simulink library "outp"  (R2021b)
settings: Solver=VariableStepAuto  StartTime=0.0  StopTime=10.0  RelTol=1e-3
undefined symbols (not defined in the file or in its folder): ENUM_PMMMODE_CHARGE, ENUM_PMMMODE_IDLE, ENUM_PMMMODE_INITIALIZE, ENUM_PMMMODE_POWERDOWN, ENUM_PMMMODE_SLEEP, Left, outp, slcm, TRUE
libraries: FVT_lib x645, hcu_lib x4, simulink x1
(part 4 of 7)

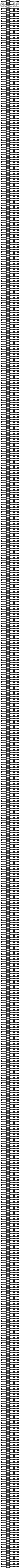
== system outp/OUTP/outpmodule ==
  VACC_HVTHCMSysAvail_enum : Inport
  VACC_LVBattVoltSta_enum : Inport  Port=2
  VACC_VehHVPwrAvail4THCM_W : Inport  Port=3
  VACC_EHPSEnDem_enum : Inport  Port=4
  VACC_CACPresWarnSta_flg : Inport  Port=5
  VACC_CACTempWarnSta_flg : Inport  Port=6
  VACC_EACEnDem_enum : Inport  Port=7
  VAPM_VehSpeedToAPM_kph : Inport  Port=8
  VAPM_VehSpeedTimeOut_flg : Inport  Port=9
  VAPM_FSOffSw_enum : Inport  Port=10
  VAPM_FSOffSwTimeOut_flg : Inport  Port=11
  VAPM_ChrgPlugSta_enum : Inport  Port=12
  VAPM_PASDRMR_cm : Inport  Port=13
  VAPM_PASDRML_cm : Inport  Port=14
  VAPM_PASDRCR_cm : Inport  Port=15
  VAPM_PASDRCL_cm : Inport  Port=16
  VAPM_PASDFMR_cm : Inport  Port=17
  VAPM_PASDFML_cm : Inport  Port=18
  VAPM_PASDFCR_cm : Inport  Port=19
  VAPM_PASDFCL_cm : Inport  Port=20
  VAPM_APSDRLR_cm : Inport  Port=21
  VAPM_APSDRLL_cm : Inport  Port=22
  VAPM_APSDFLR_cm : Inport  Port=23
  VAPM_APSDFLL_cm : Inport  Port=24
  VAPM_PASAFCL_enum : Inport  Port=25
  VAPM_PASARMR_enum : Inport  Port=26
  VAPM_PASARML_enum : Inport  Port=27
  VAPM_PASARCR_enum : Inport  Port=28
  VAPM_PASARCL_enum : Inport  Port=29
  VAPM_PASAFMR_enum : Inport  Port=30
  VAPM_PASAFML_enum : Inport  Port=31
  VAPM_PASAFCR_enum : Inport  Port=32
  VAPM_USSStaRMR_flg : Inport  Port=33
  VAPM_USSStaRML_flg : Inport  Port=34
  VAPM_USSStaRLR_flg : Inport  Port=35
  VAPM_USSStaRLL_flg : Inport  Port=36
  VAPM_USSStaRCR_flg : Inport  Port=37
  VAPM_USSStaRCL_flg : Inport  Port=38
  VAPM_USSStaFMR_flg : Inport  Port=39
  VAPM_USSStaFML_flg : Inport  Port=40
  VAPM_USSStaFLR_flg : Inport  Port=41
  VAPM_USSStaFLL_flg : Inport  Port=42
  VAPM_USSStaFCR_flg : Inport  Port=43
  VAPM_USSStaFCL_flg : Inport  Port=44
  VAPM_Chime_enum : Inport  Port=45
  VAPM_SNSRLayout_enum : Inport  Port=46
  VAPM_StaFSya_flg : Inport  Port=47
  VAPM_ModOperation_enum : Inport  Port=48
  VAPM_BrkPedalPosToAPM_pct : Inport  Port=49
  VAPM_BrkPedalPosTimeOut_flg : Inport  Port=50
  VAPM_LFRawWhlSpeed_kph : Inport  Port=51
  VAPM_LFRawWhlSpeedTimeOut_flg : Inport  Port=52
  VAPM_RFRawWhlSpeed_kph : Inport  Port=53
  VAPM_RFRawWhlSpeedTimeOut_flg : Inport  Port=54
  VAPM_LRRawWhlSpeed_kph : Inport  Port=55
  VAPM_LRRawWhlSpeedTimeOut_flg : Inport  Port=56
  VAPM_RRRawWhlSpeed_kph : Inport  Port=57
  VAPM_RRRawWhlSpeedTimeOut_flg : Inport  Port=58
  VAPM_LFRawWhlSpeedV_flg : Inport  Port=59
  VAPM_LFRawWhlSpeedVTimeOut_flg : Inport  Port=60
  VAPM_RFRawWhlSpeedV_flg : Inport  Port=61
  VAPM_RFRawWhlSpeedVTimeOut_flg : Inport  Port=62
  VAPM_LRRawWhlSpeedV_flg : Inport  Port=63
  VAPM_LRRawWhlSpeedVTimeOut_flg : Inport  Port=64
  VAPM_RRRawWhlSpeedV_flg : Inport  Port=65
  VAPM_RRRawWhlSpeedVTimeOut_flg : Inport  Port=66
  VAPM_LFWhlRotDir_enum : Inport  Port=67
  VAPM_LFWhlRotDirTimeOut_flg : Inport  Port=68
  VAPM_RFWhlRotDir_enum : Inport  Port=69
  VAPM_RFWhlRotDirTimeOut_flg : Inport  Port=70
  VAPM_LRWhlRotDir_enum : Inport  Port=71
  VAPM_LRWhlRotDirTimeOut_flg : Inport  Port=72
  VAPM_RRWhlRotDir_enum : Inport  Port=73
  VAPM_RRWhlRotDirTimeOut_flg : Inport  Port=74
  VAPM_LFPulseCountV_flg : Inport  Port=75
  VAPM_LFPulseCountVTimeOut_flg : Inport  Port=76
  VAPM_RFPulseCountV_flg : Inport  Port=77
  VAPM_RFPulseCountVTimeOut_flg : Inport  Port=78
  VAPM_LRPulseCountV_flg : Inport  Port=79
  VAPM_LRPulseCountVTimeOut_flg : Inport  Port=80
  VAPM_RRPulseCountV_flg : Inport  Port=81
  VAPM_RRPulseCountVTimeOut_flg : Inport  Port=82
  VAPM_LFPulseCount_enum : Inport  Port=83
  VAPM_LFPulseCountTimeOut_flg : Inport  Port=84
  VAPM_RFPulseCount_enum : Inport  Port=85
  VAPM_RFPulseCountTimeOut_flg : Inport  Port=86
  VAPM_LRPulseCount_enum : Inport  Port=87
  VAPM_LRPulseCountTimeOut_flg : Inport  Port=88
  VAPM_RRPulseCount_enum : Inport  Port=89
  VAPM_RRPulseCountTimeOut_flg : Inport  Port=90
  VAPM_ShifterHandleCmd_enum : Inport  Port=91
  VAPM_ShifterHandleCmdTimeOut_flg : Inport  Port=92
  VAPM_DriIntend_enum : Inport  Port=93
  VAPM_DriIntendTimeOut_flg : Inport  Port=94
  VAPM_EPSAOIControl_enum : Inport  Port=95
  VAPM_EPSAOIControlTimeOut_flg : Inport  Port=96
  VAPM_SASAngle_Deg : Inport  Port=97
  VAPM_SASAngleTimeOut_flg : Inport  Port=98
  VAPM_SASSpeed_degps : Inport  Port=99
  VAPM_SASSpeedTimeOut_flg : Inport  Port=100
  VAPM_SASSpeedValid_flg : Inport  Port=101
  VAPM_SASSpeedValidTimeOut_flg : Inport  Port=102
  VAPM_SASCAL_flg : Inport  Port=103
  VAPM_SASCALTimeOut_flg : Inport  Port=104
  VAPM_SASV_flg : Inport  Port=105
  VAPM_SASVTimeOut_flg : Inport  Port=106
  VAPM_GRADE_Deg : Inport  Port=107
  VAPM_GRADETimeOut_flg : Inport  Port=108
  VAPM_YawRate_degps : Inport  Port=109
  VAPM_YawRateTimeOut_flg : Inport  Port=110
  VAPM_LatAccel_Gps : Inport  Port=111
  VAPM_LatAccelTimeOut_flg : Inport  Port=112
  VAPM_LongAccel_Gps : Inport  Port=113
  VAPM_LongAccelTimeOut_flg : Inport  Port=114
  VAPM_MCPressure_bar : Inport  Port=115
  VAPM_MCPressureTimeOut_flg : Inport  Port=116
  VAPM_YawRateV_flg : Inport  Port=117
  VAPM_YawRateVTimeOut_flg : Inport  Port=118
  VAPM_LatAccelV_flg : Inport  Port=119
  VAPM_LatAccelVTimeOut_flg : Inport  Port=120
  VAPM_LongAccelV_flg : Inport  Port=121
  VAPM_LongAccelVTimeOut_flg : Inport  Port=122
  VAPM_MCPressureV_bar : Inport  Port=123
  VAPM_MCPressureVTimeOut_flg : Inport  Port=124
  VAPM_BrkSwSta_flg : Inport  Port=125
  VAPM_BrkSwStaTimeOut_flg : Inport  Port=126
  VAPM_BrkSwV_flg : Inport  Port=127
  VAPM_BrkSwVTimeOut_flg : Inport  Port=128
  VAPM_ESCStandstill_flg : Inport  Port=129
  VAPM_ESCStandstillTimeOut_flg : Inport  Port=130
  VAPM_ESCAPSSta_enum : Inport  Port=131
  VAPM_ESCAPSStaTimeOut_flg : Inport  Port=132
  VAPM_EPBExtReleaseAvail_flg : Inport  Port=133
  VAPM_EPBExtReleaseAvailTimeOut_flg : Inport  Port=134
  VAPM_EPBExtApplyAvail_flg : Inport  Port=135
  VAPM_EPBExtApplyAvailTimeOut_flg : Inport  Port=136
  VAPM_EPBErrSta_enum : Inport  Port=137
  VAPM_EPBErrStaTimeOut_flg : Inport  Port=138
  VAPM_EPBSta_enum : Inport  Port=139
  VAPM_EPBStaTimeOut_flg : Inport  Port=140
  VAPM_AVMparkingcancel_enum : Inport  Port=141
  VAPM_AVMparkingcancelTimeOut_flg : Inport  Port=142
  VAPM_AVMparkingexcute_enum : Inport  Port=143
  VAPM_AVMparkingexcuteTimeOut_flg : Inport  Port=144
  VAPM_AVMParkingmode_enum : Inport  Port=145
  VAPM_AVMParkingmodeTimeOut_flg : Inport  Port=146
  VAPM_AVMErrSTA_flg : Inport  Port=147
  VAPM_AVMErrSTATimeOut_flg : Inport  Port=148
  VAPM_IVIStatus_flg : Inport  Port=149
  VAPM_IVIStatusTimeOut_flg : Inport  Port=150
  VAPM_CAASSw_enum : Inport  Port=151
  VAPM_CAASSwTimeOut_flg : Inport  Port=152
  VAPM_IVIScreen_enum : Inport  Port=153
  VAPM_IVIScreenTimeOut_flg : Inport  Port=154
  VAPM_ABSActiveToAPM_flg : Inport  Port=155
  VAPM_ABSActiveTimeOut_flg : Inport  Port=156
  VAPM_TCSActiveToAPM_flg : Inport  Port=157
  VAPM_TCSActiveTimeOut_flg : Inport  Port=158
  VAPM_DriverSeatBeltCmd_flg : Inport  Port=159
  VAPM_DriverSeatBeltCmdTimeOut_flg : Inport  Port=160
  VAPM_APSProgressPCT_pct : Inport  Port=161
  VAPM_APSRQDisplay_enum : Inport  Port=162
  VAPM_APSSWVer_enum : Inport  Port=163
  VAPM_APSHWVer_enum : Inport  Port=164
  VAPM_APSExitCondition_enum : Inport  Port=165
  VAPM_APSAngleTarget_Deg : Inport  Port=166
  VAPM_APSVRqEPASCtrl_flg : Inport  Port=167
  VAPM_APSRqEPASCtrl_flg : Inport  Port=168
  VAPM_CAASSta_enum : Inport  Port=169
  VBCM_HornCtrl_flg : Inport  Port=170
  VBCM_FRHaltBrakeSta_enum : Inport  Port=171
  VBCM_FRDisIntEmCmd_flg : Inport  Port=172
  VBCM_FROpenClosePBCmd_enum : Inport  Port=173
  VBCM_DoorStaSta_enum : Inport  Port=174
  VBCM_BrakeLamp_flg : Inport  Port=175
  VBCM_LDRL_flg : Inport  Port=176
  VBCM_RDRL_flg : Inport  Port=177
  VBCM_ReverseLamp_flg : Inport  Port=178
  VBCM_RrFogLamp_flg : Inport  Port=179
  VBCM_HBeam_flg : Inport  Port=180
  VBCM_LBeam_flg : Inport  Port=181
  VBCM_PosLamp_flg : Inport  Port=182
  VBCM_HazardSW_flg : Inport  Port=183
  VBCM_LTurnLP_flg : Inport  Port=184
  VBCM_RTurnLP_flg : Inport  Port=185
  VBCM_LSMLPCmd_flg : Inport  Port=186
  VBCM_RSMLPCmd_flg : Inport  Port=187
  VBCM_TurnLpLActiveCmd_flg : Inport  Port=188
  VBCM_TurnLpRActiveCmd_flg : Inport  Port=189
  VBCM_BBuzzerCmd_flg : Inport  Port=190
  VBCM_FrWiperL_flg : Inport  Port=191
  VBCM_FrWiperH_flg : Inport  Port=192
  VBCM_WasherCtrl_enum : Inport  Port=193
  VBCM_RrRmLampBrightCmd_enum : Inport  Port=194
  VBCM_WelcomeDemoSta_flg : Inport  Port=195
  VBCM_FrAtmoLampCmd_flg : Inport  Port=196
  VBCM_RrAtmoLampCmd_flg : Inport  Port=197
  VBCM_TgateHDSWLSta_flg : Inport  Port=198
  VBCM_TgateHDSWRSta_flg : Inport  Port=199
  VBCM_TgateSWLSta_flg : Inport  Port=200
  VBCM_TgateSWRSta_flg : Inport  Port=201
  VBCM_LTgateRelCmd_flg : Inport  Port=202
  VBCM_RTgateRelCmd_flg : Inport  Port=203
  VBCM_FDDoorOpen_enum : Inport  Port=204
  VBCM_FDDoorstate_enum : Inport  Port=205
  VDHP_ActAPSPosn_pct : Inport  Port=206
  VDHP_EAPS1MIN_pct : Inport  Port=207
  VDHP_EAPS2MIN_pct : Inport  Port=208
  VDKC_DKCTimeSN_cnt : Inport  Port=209
  VDKC_DKCAuthSta_enum : Inport  Port=210
  VDSC_DISCTurn_flg : Inport  Port=211
  VDSC_DISCTargetSpd_kph : Inport  Port=212
  VDSC_DISCSta_enum : Inport  Port=213
  VDSC_DISCButtSta_flg : Inport  Port=214
  VNMM_AllCANTxReq_flg : Inport  Port=215
  VNMM_NMmTxReq_flg : Inport  Port=216
  VNMM_Awake_enum : Inport  Port=217
  VNMM_CSB_flg : Inport  Port=218
  VNMM_ErrorState_enum : Inport  Port=219
  VNMM_NodeID_enum : Inport  Port=220
  VNMM_PNI_flg : Inport  Port=221
  VNMM_RptMsgReq_flg : Inport  Port=222
  VNMM_WakeUp_enum : Inport  Port=223
  VNMM_ActiveWU_flg : Inport  Port=224
  VNMM_SysNMmSta_enum : Inport  Port=225
  VNMM_NetworkReq_flg : Inport  Port=226
  VPMM_PowerUpState_enum : Inport  Port=227
  VPMM_PowerDownState_enum : Inport  Port=228
  VPMM_PowerUpFault_enum : Inport  Port=229
  VPMM_PowerDownFault_enum : Inport  Port=230
  VPMM_ActiveDischargeReq_flg : Inport  Port=231
  VPMM_DCDCEnaReq_flg : Inport  Port=232
  VPMM_DCDCVoltSetpoint_V : Inport  Port=233
  VPMM_HVBatCnctReq_flg : Inport  Port=234
  VPMM_HVSysReadyToCharge_enum : Inport  Port=235
  VPMM_PowerSta_enum : Inport  Port=236
  VPMM_LVPwrSta_flg : Inport  Port=237
  VPMM_HVPwrSta_flg : Inport  Port=238
  VPMM_SysPowerMode_enum : Inport  Port=239
  VPMM_FrMCUEnaReq_flg : Inport  Port=240
  VPMM_RrMCUEnaReq_flg : Inport  Port=241
  VPMM_DrivetrainSelect_enum : Inport  Port=242
  VPMM_DrSeatSta_enum : Inport  Port=243
  VPMM_PwrStaSelect_enum : Inport  Port=244
  VPMM_PwrStaConstraint_enum : Inport  Port=245
  VPMM_TCountSta_enum : Inport  Port=246
  VPMM_PwrUpReq_enum : Inport  Port=247
  VPMM_PwrDownReq_enum : Inport  Port=248
  VPMM_LowSOCWarn_enum : Inport  Port=249
  VPMM_ReVehThdChkSta_enum : Inport  Port=250
  VPMM_LVSysErrPwrOutErr_flg : Inport  Port=251
  VPMM_EvccAplusPwrUpReq_flg : Inport  Port=252
  VPMM_PwrStaONTOPopReq_flg : Inport  Port=253
  VPMM_IVIPwrStaONTOPopT_s : Inport  Port=254
  VPMM_LVChrgHoldTtimer_s : Inport  Port=255
  VPMM_LVBattChrgTimeCnt_s : Inport  Port=256
  VPMM_SilentChkAllowSleep_flg : Inport  Port=257
  VPMM_TimerAllowSleep_flg : Inport  Port=258
  VPMM_FDADC12VDetAvg_mV : Inport  Port=259
  VPMM_PMMAllowECUSleep_flg : Inport  Port=260
  VPMM_LVSilentChrgSta_enum : Inport  Port=261
  VPMM_LVSilentChrgReq_flg : Inport  Port=262
  VPMM_LVSilentChrgLv_enum : Inport  Port=263
  VPMM_CtrlFrPwrStbA1P_flg : Inport  Port=264
  VPMM_CtrlFrRC1_flg : Inport  Port=265
  VPMM_CtrlFrBMSCCUCIR_flg : Inport  Port=266
  VPMM_CtrlFrEDUINVERTER_flg : Inport  Port=267
  VPMM_HWResetSta_enum : Inport  Port=268
  VPMM_CtrlDrPwrStbA2_flg : Inport  Port=269
  VPMM_PwrStaTOSta_enum : Inport  Port=270
  VPMM_DCDCRlyDem_enum : Inport  Port=271
  VPMM_EACRlyDem_enum : Inport  Port=272
  VPMM_EHPSRlyDem_enum : Inport  Port=273
  VPMM_DCDCEnDem_enum : Inport  Port=274
  VSCP_Vehspeed_kph : Inport  Port=275
  VSCP_SCPBrkSwSta_flg : Inport  Port=276
  VSCP_AmberWnlmpSta_flg : Inport  Port=277
  VSCP_ABSWnlmpSta_flg : Inport  Port=278
  VSCP_HSAFailed_flg : Inport  Port=279
  VSCP_MeterIndVehSpeed_kph : Inport  Port=280
  VSCP_ABSFailed_flg : Inport  Port=281
  VSCP_ABSActive_flg : Inport  Port=282
  VSCP_HSAActive_flg : Inport  Port=283
  VSCP_RedWnlmpSta_flg : Inport  Port=284
  VSCP_BrkPedalPos_pct : Inport  Port=285
  VSCP_OpenStatusOfDoor1_enum : Inport  Port=286
  VSCP_OpenStatusOfDoor2_enum : Inport  Port=287
  VSCP_SeatBeltSwitch_enum : Inport  Port=288
  VSCP_triggerBAM_flg : Inport  Port=289
  VSCP_CFGEM1Ctrl_raw : Inport  Port=290
  VSCP_CFGEM1BAMTSize_raw : Inport  Port=291
  VSCP_CFGEM1BAMTNum_raw : Inport  Port=292
  VSCP_CFGEM1BAMRsv_raw : Inport  Port=293
  VSCP_CFGEM1BAMPGN_raw : Inport  Port=294
  VSCP_triggerDT_flg : Inport  Port=295
  VSCP_DTbyte0_raw : Inport  Port=296
  VSCP_DTbyte1_raw : Inport  Port=297
  VSCP_DTbyte2_raw : Inport  Port=298
  VSCP_DTbyte3_raw : Inport  Port=299
  VSCP_DTbyte4_raw : Inport  Port=300
  VSCP_DTbyte5_raw : Inport  Port=301
  VSCP_DTbyte6_raw : Inport  Port=302
  VSCP_DTbyte7_raw : Inport  Port=303
  VSYS_HWVer1_cnt : Inport  Port=304
  VSYS_HWVer2_cnt : Inport  Port=305
  VSYS_HWVer3_cnt : Inport  Port=306
  VSYS_CarModel1_cnt : Inport  Port=307
  VSYS_CarModel2_cnt : Inport  Port=308
  VSYS_CarModel3_cnt : Inport  Port=309
  VSYS_ECU1_cnt : Inport  Port=310
  VSYS_ECU2_cnt : Inport  Port=311
  VSYS_Major1_cnt : Inport  Port=312
  VSYS_Major2_cnt : Inport  Port=313
  VSYS_Minor1_cnt : Inport  Port=314
  VSYS_Minor2_cnt : Inport  Port=315
  VSYS_Patch1_cnt : Inport  Port=316
  VSYS_Patch2_cnt : Inport  Port=317
  VSYS_Country1_cnt : Inport  Port=318
  VSYS_Country2_cnt : Inport  Port=319
  VSYS_Variation_cnt : Inport  Port=320
  VSYS_Dash1_cnt : Inport  Port=321
  VSYS_Change1_cnt : Inport  Port=322
  VSYS_Change2_cnt : Inport  Port=323
  VSYS_Dash2_cnt : Inport  Port=324
  VSYS_SHA1_cnt : Inport  Port=325
  VSYS_SHA2_cnt : Inport  Port=326
  VSYS_SHA3_cnt : Inport  Port=327
  VSYS_SHA4_cnt : Inport  Port=328
  VSYS_SHA5_cnt : Inport  Port=329
  VSYS_SHA6_cnt : Inport  Port=330
  VSYS_SHA7_cnt : Inport  Port=331
  VSYS_SHA8_cnt : Inport  Port=332
  VSYS_NvWriteReqRisingEdge_flg : Inport  Port=333
  VSYS_FdcSlpReqRisingEdge_flg : Inport  Port=334
  VSYS_FdcSlpTime_sec : Inport  Port=335
  VSYS_PmicBootReason_enum : Inport  Port=336
  VSYS_WisrBootReason_raw32 : Inport  Port=337
  VSYS_AcoreRebootCmdACK_flg : Inport  Port=338
  VSYS_CurrentNmState_enum : Inport  Port=339
  VTHC_FDCompCmd_rpm : Inport  Port=340
  VTHC_FDSOV1Cmd_flg : Inport  Port=341
  VTHC_FDSOV2Cmd_flg : Inport  Port=342
  VTHC_FDSOV3Cmd_flg : Inport  Port=343
  VTHC_FDEXV1Cmd_step : Inport  Port=344
  VTHC_FDEXV2Cmd_step : Inport  Port=345
  VTHC_FDSOTXVCmd_flg : Inport  Port=346
  VTHC_FDFWVCmd_flg : Inport  Port=347
  VTHC_FDTWVCmd_pct : Inport  Port=348
  VTHC_FDFrWPTCHeatPwrCmd_W : Inport  Port=349
  VTHC_CoolgFanActDuty_pct : Inport  Port=350
  VTHC_FDAGSCmd_enum : Inport  Port=351
  VTHC_FDEWP1Cmd_enum : Inport  Port=352
  VTHC_FDEWP2Cmd_enum : Inport  Port=353
  VTHC_FDEWP3Cmd_enum : Inport  Port=354
  VTHC_FDFrLeAPTCHeatPwrCmd_W : Inport  Port=355
  VTHC_FDFrRiAPTCHeatPwrCmd_W : Inport  Port=356
  VTHC_FDRrAPTCHeatPwrCmd_W : Inport  Port=357
  VTHC_FDBlowerCmd_pct : Inport  Port=358
  VTHC_BatteryMode_enum : Inport  Port=359
  VTHC_EDriveMode_enum : Inport  Port=360
  VTHC_CabinMode_enum : Inport  Port=361
  VTHC_CCUACLampSts_flg : Inport  Port=362
  VTHC_CCUAutoLampSts_flg : Inport  Port=363
  VTHC_CCUACMaxLampSts_flg : Inport  Port=364
  VTHC_CCUSyncLampSts_flg : Inport  Port=365
  VTHC_sigAirIntenZon1St_enum : Inport  Port=366
  VTHC_sigWindDirZon1St_enum : Inport  Port=367
  VTHC_sigRecircSt_flg : Inport  Port=368
  VTHC_sigSetTempZon1St_C : Inport  Port=369
  VTHC_sigSetTempZon2St_C : Inport  Port=370
  VTHC_sigClntTHvBattOut_C : Inport  Port=371
  VTHC_sigCbnSolarLeft_W : Inport  Port=372
  VTHC_sigClntTHvBattIn_C : Inport  Port=373
  VTHC_sigCbnSolarRight_W : Inport  Port=374
  VTHC_sigAmbAirT_C : Inport  Port=375
  VTHC_sigCbnAirT_C : Inport  Port=376
  VTHC_ACSubMode_enum : Inport  Port=377
  VTHC_FDRecyAutoCmd_enum : Inport  Port=378
  VTHC_ACModeMem_enum : Inport  Port=379
  VTHC_Face_flg : Inport  Port=380
  VTHC_Foot_flg : Inport  Port=381
  VTHC_Frost_flg : Inport  Port=382
  VTHC_FaceM_flg : Inport  Port=383
  VTHC_FootM_flg : Inport  Port=384
  VTHC_CCUSyncSts_flg : Inport  Port=385
  VTHC_ACForceOFF_flg : Inport  Port=386
  VTHC_RecAutoFlg_flg : Inport  Port=387
  VTHC_AirIntenZone1M_enum : Inport  Port=388
  VTHC_fdefog_flg : Inport  Port=389
  VTHC_sigSetTempZon2StM_C : Inport  Port=390
  VTHC_FDCTHCMAPTCWarningSta_flg : Inport  Port=391
  VTPM_LFBatWarn_flg : Inport  Port=392
  VTPM_RFBatWarn_flg : Inport  Port=393
  VTPM_LRBatWarn_flg : Inport  Port=394
  VTPM_RRBatWarn_flg : Inport  Port=395
  VTPM_LFWheelPress_raw8 : Inport  Port=396
  VTPM_RFWheelPress_raw8 : Inport  Port=397
  VTPM_LRWheelPress_raw8 : Inport  Port=398
  VTPM_RRWheelPress_raw8 : Inport  Port=399
  VTPM_LFWheelTemp_C : Inport  Port=400
  VTPM_RFWheelTemp_C : Inport  Port=401
  VTPM_LRWheelTemp_C : Inport  Port=402
  VTPM_RRWheelTemp_C : Inport  Port=403
  VTPM_LFSensorFail_flg : Inport  Port=404
  VTPM_RFSensorFail_flg : Inport  Port=405
  VTPM_LRSensorFail_flg : Inport  Port=406
  VTPM_RRSensorFail_flg : Inport  Port=407
  VTPM_LFWheelDebug_flg : Inport  Port=408
  VTPM_LRWheelDebug_flg : Inport  Port=409
  VTPM_RFWheelDebug_flg : Inport  Port=410
  VTPM_RRWheelDebug_flg : Inport  Port=411
  VTPM_TPMSResButtAllow_flg : Inport  Port=412
  VTPM_TPMSCaliButtAllow_flg : Inport  Port=413
  VTPM_LFPressIndi_enum : Inport  Port=414
  VTPM_RFPressIndi_enum : Inport  Port=415
  VTPM_LRPressIndi_enum : Inport  Port=416
  VTPM_RRPressIndi_enum : Inport  Port=417
  VTPM_TPMSWarnIndi_enum : Inport  Port=418
  VTPM_LFWheelTmpIndi_flg : Inport  Port=419
  VTPM_RFWheelTmpIndi_flg : Inport  Port=420
  VTPM_LRWheelTmpIndi_flg : Inport  Port=421
  VTPM_RRWheelTmpIndi_flg : Inport  Port=422
  VTPM_LFWheelPSW_raw8 : Inport  Port=423
  VTPM_LRWheelPSW_raw8 : Inport  Port=424
  VTPM_RFWheelPSW_raw8 : Inport  Port=425
  VTPM_RRWheelPSW_raw8 : Inport  Port=426
  VTPM_CWheelTips_enum : Inport  Port=427
  VTPM_AutoLTips_enum : Inport  Port=428
  VTPM_LFSensorMode_flg : Inport  Port=429
  VTPM_RFSensorMode_flg : Inport  Port=430
  VTPM_LRSensorMode_flg : Inport  Port=431
  VTPM_RRSensorMode_flg : Inport  Port=432
  VTPM_S1ID_raw32 : Inport  Port=433
  VTPM_S2ID_raw32 : Inport  Port=434
  VTPM_S3ID_raw32 : Inport  Port=435
  VTPM_S4ID_raw32 : Inport  Port=436
  VTPM_S1L_enum : Inport  Port=437
  VTPM_S2L_enum : Inport  Port=438
  VTPM_S3L_enum : Inport  Port=439
  VTPM_S4L_enum : Inport  Port=440
  VTPM_ALFin_flg : Inport  Port=441
  VTPM_LFP20_raw8 : Inport  Port=442
  VTPM_RFP20_raw8 : Inport  Port=443
  VTPM_LRP20_raw8 : Inport  Port=444
  VTPM_RRP20_raw8 : Inport  Port=445
  VTPM_FAT_flg : Inport  Port=446
  VTPM_IDin_raw32 : Inport  Port=447
  VTPM_S1WheelDebugALTU_pct : Inport  Port=448
  VTPM_S2WheelDebugALTU_pct : Inport  Port=449
  VTPM_S3WheelDebugALTU_pct : Inport  Port=450
  VTPM_S4WheelDebugALTU_pct : Inport  Port=451
  VTPM_ID1messageALTU_raw8 : Inport  Port=452
  VTPM_ID2messageALTU_raw8 : Inport  Port=453
  VTPM_ID3messageALTU_raw8 : Inport  Port=454
  VTPM_ID4messageALTU_raw8 : Inport  Port=455
  VTPM_Chkfin_flg : Inport  Port=456
  VTPM_SetIDLoc_flg : Inport  Port=457
  VTPM_TPMSStorge_flg : Inport  Port=458
  VTPM_ChkStorge_flg : Inport  Port=459
  VTPM_TPMSResButt_flg : Inport  Port=460
  VTPM_LFPindi_enum : Inport  Port=461
  VTPM_RFPind_enum : Inport  Port=462
  VTPM_LRPindi_enum : Inport  Port=463
  VTPM_RRPindi_enum : Inport  Port=464
  VTPM_WriteChkLFID_raw : Inport  Port=465
  VTPM_WriteChkRFID_raw : Inport  Port=466
  VTPM_WriteChkLRID_raw : Inport  Port=467
  VTPM_WriteChkRRID_raw : Inport  Port=468
  VTPM_WriteChkfinLFID_raw : Inport  Port=469
  VTPM_WriteChkfinRFID_raw : Inport  Port=470
  VTPM_WriteChkfinLRID_raw : Inport  Port=471
  VTPM_WriteChkfinRRID_raw : Inport  Port=472
  VTPM_Flashchkdatavalid_enum : Inport  Port=473
  VTPM_Flashdatavalid_enum : Inport  Port=474
  VTPM_unlearnSfali_flg : Inport  Port=475
  VTPM_unlearnSfailvalid_enum : Inport  Port=476
  VTPM_Prepresstempvalid_enum : Inport  Port=477
  VTPM_FlashS1ID_raw : Inport  Port=478
  VTPM_FlashS2ID_raw : Inport  Port=479
  VTPM_FlashS3ID_raw : Inport  Port=480
  VTPM_FlashS4ID_raw : Inport  Port=481
  VTPM_FlashIDvalid_enum : Inport  Port=482
  VTQD_ParkRequest_flg : Inport  Port=483
  VTQD_TqSourceFr_enum : Inport  Port=484
  VTQD_TqSourceRr_enum : Inport  Port=485
  VTQD_FrEDUAvailBrkRgnTq_Nm : Inport  Port=486
  VTQD_RrEDUAvailBrkRgnTq_Nm : Inport  Port=487
  VTQD_EVDriveMode_enum : Inport  Port=488
  VTQD_ShiftGearPosn_enum : Inport  Port=489
  VTQD_PButtonSta_enum : Inport  Port=490
  VTQD_FrActvDmpDisabReq_flg : Inport  Port=491
  VTQD_RrActvDmpDisabReq_flg : Inport  Port=492
  VTQD_FrRgnDecrSta_flg : Inport  Port=493
  VTQD_RrRgnDecrSta_flg : Inport  Port=494
  VTQD_DriverWhlTqDemFr_Nm : Inport  Port=495
  VTQD_DriverWhlTqDemRr_Nm : Inport  Port=496
  VTQD_FrEDUActTq_Nm : Inport  Port=497
  VTQD_RrEDUActTq_Nm : Inport  Port=498
  VTQD_FrEDURolRgnTq_Nm : Inport  Port=499
  VTQD_RrEDURolRgnTq_Nm : Inport  Port=500
  VTQD_FrEDUSpd_rpm : Inport  Port=501
  VTQD_RrEDUSpd_rpm : Inport  Port=502
  VTQD_FrEDUSpdValid_flg : Inport  Port=503
  VTQD_FrEDUAvailBrkRgnTqV_flg : Inport  Port=504
  VTQD_RrEDUSpdValid_flg : Inport  Port=505
  VTQD_RrEDUAvailBrkRgnTqV_flg : Inport  Port=506
  VTQD_RgnAbnorSta_flg : Inport  Port=507
  VTQD_PTCSPermSta_flg : Inport  Port=508
  VTQD_FrRgnPermSta_flg : Inport  Port=509
  VTQD_RrRgnPermSta_flg : Inport  Port=510
  VTQD_FrIdcMin_A : Inport  Port=511
  VTQD_FrIdcMax_A : Inport  Port=512
  VTQD_FrUdcMin_V : Inport  Port=513
  VTQD_FrUdcMax_V : Inport  Port=514
  VTQD_RrIdcMin_A : Inport  Port=515
  VTQD_RrIdcMax_A : Inport  Port=516
  VTQD_RrUdcMin_V : Inport  Port=517
  VTQD_RrUdcMax_V : Inport  Port=518
  VTQD_ReBrakeLPReq_flg : Inport  Port=519
  VTQD_CreepON_flg : Inport  Port=520
  VTQD_ActEMpTrq_pct : Inport  Port=521
  VTQD_ActMaxAvaEMRecpTrq_pct : Inport  Port=522
  VTQD_ActDriveDirect_enum : Inport  Port=523
  VTQD_DLEngaged_enum : Inport  Port=524
  VTQD_EMTrqModeDrvBrk_enum : Inport  Port=525
  VTQD_ActEMpTrqHrls_pct : Inport  Port=526
  VTQD_ActEMOutSftSpd_rpm : Inport  Port=527
  VTQD_DrvDemEMRtapTrq_pct : Inport  Port=528
  VTQD_SACtrlDev_enum : Inport  Port=529
  VTQD_RetSelNonEng_pct : Inport  Port=530
  VTQD_ShiftPgs_enum : Inport  Port=531
  VTQD_AccPedal1LowSW_enum : Inport  Port=532
  VTQD_AccPedalPos1_pct : Inport  Port=533
  VTQD_ParkBrakeSW_enum : Inport  Port=534
  VTQD_VCUVehSpd_kph : Inport  Port=535
  VTQD_BrakeSW_enum : Inport  Port=536
  VTQD_NFricPercTorq_pct : Inport  Port=537
  VTQD_EMParasLoss_pct : Inport  Port=538
  VTQD_EEC2MSGCnt_raw : Inport  Port=539
  VTQD_EEC2MSGCS_raw : Inport  Port=540
  VTQD_FDCCHAEBSRd4BRSta_enum : Inport  Port=541
  VTQD_FDCCHAEBSHBSwSta_enum : Inport  Port=542
  VTQD_FDCCHAEBSHHSwSta_enum : Inport  Port=543
  VTQD_FDCVCUTUpAStaSta_enum : Inport  Port=544
  VTQD_FDCVCUDACStatusSta_enum : Inport  Port=545
  VTQR_FrTMTqReq_Nm : Inport  Port=546
  VTQR_RrTMTqReq_Nm : Inport  Port=547
  VV2L_ReqOBCV2LEna_enum : Inport  Port=548
  VV2L_ReqV2LIVIPopup_enum : Inport  Port=549
  VVMC_FeatSetSpdFinal_raw32 : Inport  Port=550
  VVMC_VehicleSpeed_mph : Inport  Port=551
  VVMC_VehicleSpeed_kph : Inport  Port=552
  VVMC_MeterIndSpeed_raw32 : Inport  Port=553
  VVMC_VMCAEBCtrlAvail_flg : Inport  Port=554
  VVMC_VMCACCCtrlAvail_flg : Inport  Port=555
  VVMC_VMCCCCtrlAvail_flg : Inport  Port=556
  VVMC_VMCMSACtrlAvail_flg : Inport  Port=557
  VVMC_FeatArbitrSta_enum : Inport  Port=558
  VVMC_FeatReqSpd_kph : Inport  Port=559
  VVMC_JerkPCT_pct : Inport  Port=560
  VVMC_LimitPCT_pct : Inport  Port=561
  VVMC_FrontRearSlipRatioCtrl_flg : Inport  Port=562
  VVMC_RearWhlSlipRatioCtrl_flg : Inport  Port=563
  VVMC_SingleWhlSlipRatioCtrl_flg : Inport  Port=564
  VVMC_LatAccCtrl_flg : Inport  Port=565
  VVMC_SafetyCtrl_flg : Inport  Port=566
  VVMC_SPD2ACCAct_flg : Inport  Port=567
  VVMC_AccCalcuPID_mps2 : Inport  Port=568
  VVMC_ISOAccLimit_mps2 : Inport  Port=569
  VVMC_ISODecLimit_mps2 : Inport  Port=570
  VVMC_ISOJerkLimit_mps3 : Inport  Port=571
  VVMC_ACCRequiredAccel_mps2 : Inport  Port=572
  VVMC_DISCReqAcc_mps2 : Inport  Port=573
  VVMC_FeatArbitrFinal_enum : Inport  Port=574
  VVMC_LateralCtrl_flg : Inport  Port=575
  VVMC_ADASLKASta_enum : Inport  Port=576
  VVMC_LKAStrToqReq_Nm : Inport  Port=577
  VVMC_LKATOIFault_flg : Inport  Port=578
  VVMC_LKATOIAct_enum : Inport  Port=579
  VVMC_ADASAEBReq_enum : Inport  Port=580
  VVMC_ADASFaultSta_flg : Inport  Port=581
  VVMC_AEBVehHoldReq_flg : Inport  Port=582
  VVMC_ACCVehHoldReq_flg : Inport  Port=583
  VVMC_ADASDBSReq_enum : Inport  Port=584
  VVMC_ADASACCSta_enum : Inport  Port=585
  VVMC_ACCObjDist_m : Inport  Port=586
  VVMC_ACCObjRelSpd_mps : Inport  Port=587
  VVMC_TimeGapLevel_enum : Inport  Port=588
  VVMC_ACCJerkUpperLimit_mps3 : Inport  Port=589
  VVMC_ACCComfortBandUpper_mps2 : Inport  Port=590
  VVMC_ACCJerkLowerLimit_mps3 : Inport  Port=591
  VVMC_ACCComfortBandLower_mps2 : Inport  Port=592
  VVMC_ADASVehSpdLim_raw32 : Inport  Port=593
  VVMC_ADASShftPosnReqA_flg : Inport  Port=594
  VVMC_ADASShftPosnReq_enum : Inport  Port=595
  VVMC_ADASForceIdle_flg : Inport  Port=596
  VVMC_HazardWarningReq_flg : Inport  Port=597
  VVMC_RightTurnLightReq_flg : Inport  Port=598
  VVMC_LeftTurnLightReq_flg : Inport  Port=599
  VVMC_ADASFCWSta_enum : Inport  Port=600
  VVMC_ADASLDWSta_enum : Inport  Port=601
  VVMC_ADASFltWrnReq_flg : Inport  Port=602
  VVMC_ACCObjDstLvl_enum : Inport  Port=603
  VVMC_ForceLowBeam_enum : Inport  Port=604
  VVMC_ACCTakeoverReq_flg : Inport  Port=605
  VVMC_ADASWarningMsg_enum : Inport  Port=606
  VVMC_ADASCAMSpdLim_enum : Inport  Port=607
  VVMC_TargetType_enum : Inport  Port=608
  VVMC_ADASSLIFSpdLim_enum : Inport  Port=609
  VVMC_LKAHODDisplayWarning_flg : Inport  Port=610
  VVMC_LKAHODSoundWarning_flg : Inport  Port=611
  VVMC_ADASLFCSta_enum : Inport  Port=612
  VVMC_ADASLaneModeL_enum : Inport  Port=613
  VVMC_ADASLaneModeR_enum : Inport  Port=614
  VVMC_ADASSLIFSta_enum : Inport  Port=615
  VVMC_ADASISASta_enum : Inport  Port=616
  VVMC_ADASLDWMute_flg : Inport  Port=617
  VVMC_ADASFCWMute_flg : Inport  Port=618
  VVMC_ADASLFCHandsOffWarning_enum : Inport  Port=619
  VVMC_LVDADisabled_flg : Inport  Port=620
  VVMC_LVDAMuteSta_enum : Inport  Port=621
  VVMC_LVDAFailinfo_flg : Inport  Port=622
  VVMC_LVDAWarning_flg : Inport  Port=623
  VVMC_LVDAACCStatusInformation_flg : Inport  Port=624
  VVMC_ADASLFCWarnSound_enum : Inport  Port=625
  VVMC_FCMACCmode_enum : Inport  Port=626
  VVMC_ADASLanetypeR_enum : Inport  Port=627
  VVMC_ADASLanetypeL_enum : Inport  Port=628
  VVMC_ADASLanecurveL_raw32 : Inport  Port=629
  VVMC_ADASLanecurveR_raw32 : Inport  Port=630
  VVMC_ADASAEBSta_enum : Inport  Port=631
  VVMC_FCMLDWRequest_enum : Inport  Port=632
  VVMC_FCMLDWFault_flg : Inport  Port=633
  VVMC_ACCCtrlAvail_flg : Inport  Port=634
  VVMC_ACCPedalOvrd_flg : Inport  Port=635
  VVMC_TimeGapCalcu_s : Inport  Port=636
  VVMC_CCCtrlSta_enum : Inport  Port=637
  VVMC_MSACtrlSta_enum : Inport  Port=638
  VVMC_APSCtrlAvail_flg : Inport  Port=639
  VVMC_APSStaSys_enum : Inport  Port=640
  VVMC_APSDecReqA_flg : Inport  Port=641
  VVMC_APSDecReq_mps2 : Inport  Port=642
  VVMC_APSReq_enum : Inport  Port=643
  VVMC_CCMSASpdWar_flg : Inport  Port=644
  VVMC_IMUEnaCmd_flg : Inport  Port=645
  UnitConverter{1..2,4,7,10,12..20,25..32,45..46,48,67,69,71,73,83,85,87,89,91,93,95,131,137,139,141,143,145,151,153,162..165,169,171,173..174,193..194,204..205,210,213,217,219..220,223,225,227..230,235..236,239,242..250,261,263,268,270..274,286..288,290,292..293,296..332,336,339,351..354,359..361,366..367,377..379,388,396..399,414..418,423..428,437..440,442..445,452..455,461..464,473..474,476..477,482,484..485,488..490,524..525,529,531..532,534,536,539..545,548..549,558,574,576,579..580,584..585,588,595,600..601,603..604,606..609,612..616,619,621,625..628,631..632,637..638,640,643} (236 alike) : DataTypeConversion  OutDataTypeStr=uint8
  UnitConverter{5..6,9,11,33..44,47,50,52,54,56,58..66,68,70,72,74..82,84,86,88,90,92,94,96,98,100..106,108,110,112,114,116..130,132..136,138,140,142,144,146..150,152,154..160,167..168,170,172,175..192,195..203,211,214..216,218,221..222,224,226,231..232,234,237..238,240..241,251..253,257..258,260,262,264..267,269,276..279,281..284,289,295,333..334,338,341..343,346..347,362..365,368,380..387,389,391..395,404..413,419..422,429..432,441,446,456..460,475,483,491..494,503..510,519..520,554..557,562..567,575,578,581..583,594,596..599,602,605,610..611,617..618,620,622..624,633..635,639,641,644..645} (272 alike) : DataTypeConversion  OutDataTypeStr=boolean
  UnitConverter{3,8,49,51,53,55,57,97,99,107,109,111,113,115,161,166,206..208,212,233,254..256,259,275,280,285,335,348..350,355..358,369..376,390,400..403,448..451,486..487,495..502,511..518,521..523,526..528,530,533,535,537..538,546..547,550..553,559..561,568..573,577,586..587,589..593,629..630,636,642} (109 alike) : DataTypeConversion  OutDataTypeStr=single
  UnitConverter{209,294,337,433..436,447,465..472,478..481} (20 alike) : DataTypeConversion  OutDataTypeStr=uint32
  UnitConverter{21..24,291,340,344..345} (8 alike) : DataTypeConversion  OutDataTypeStr=uint16
  VACC_CACPresWarnSta_flg_Inproc : FVT_lib/outp/OverrideAndLimit  SystemSampleTime=-1  VariantActivationTime=update diagram  Latency=0  AutoFrameSizeCalculation=off
      link override Signal_Limit/_maxval: Value=KOUTP_CACPresWarnSta_flg_maxval
      link override Signal_Limit/_minval: Value=KOUTP_CACPresWarnSta_flg_minval
      link override Signal_Override/_ovrdflg: Value=KOUTP_CACPresWarnSta_flg_ovrdflg
      link override Signal_Override/_ovrdval: Value=KOUTP_CACPresWarnSta_flg_ovrdval
  VACC_CACTempWarnSta_flg_Inproc : FVT_lib/outp/OverrideAndLimit  SystemSampleTime=-1  VariantActivationTime=update diagram  Latency=0  AutoFrameSizeCalculation=off
      link override Signal_Limit/_maxval: Value=KOUTP_CACTempWarnSta_flg_maxval
      link override Signal_Limit/_minval: Value=KOUTP_CACTempWarnSta_flg_minval
      link override Signal_Override/_ovrdflg: Value=KOUTP_CACTempWarnSta_flg_ovrdflg
      link override Signal_Override/_ovrdval: Value=KOUTP_CACTempWarnSta_flg_ovrdval
  VACC_EACEnDem_enum_Inproc : FVT_lib/outp/OverrideAndLimit  SystemSampleTime=-1  VariantActivationTime=update diagram  Latency=0  AutoFrameSizeCalculation=off
      link override Signal_Limit/_maxval: Value=KOUTP_EACEnDem_enum_maxval
      link override Signal_Limit/_minval: Value=KOUTP_EACEnDem_enum_minval
      link override Signal_Override/_ovrdflg: Value=KOUTP_EACEnDem_enum_ovrdflg
      link override Signal_Override/_ovrdval: Value=KOUTP_EACEnDem_enum_ovrdval
  VACC_EHPSEnDem_enum_Inproc : FVT_lib/outp/OverrideAndLimit  SystemSampleTime=-1  VariantActivationTime=update diagram  Latency=0  AutoFrameSizeCalculation=off
      link override Signal_Limit/_maxval: Value=KOUTP_EHPSEnDem_enum_maxval
      link override Signal_Limit/_minval: Value=KOUTP_EHPSEnDem_enum_minval
      link override Signal_Override/_ovrdflg: Value=KOUTP_EHPSEnDem_enum_ovrdflg
      link override Signal_Override/_ovrdval: Value=KOUTP_EHPSEnDem_enum_ovrdval
  VACC_HVTHCMSysAvail_enum_Inproc : FVT_lib/outp/OverrideAndLimit  SystemSampleTime=-1  VariantActivationTime=update diagram  Latency=0  AutoFrameSizeCalculation=off
      link override Signal_Limit/_maxval: Value=KOUTP_HVTHCMSysAvail_enum_maxval
      link override Signal_Limit/_minval: Value=KOUTP_HVTHCMSysAvail_enum_minval
      link override Signal_Override/_ovrdflg: Value=KOUTP_HVTHCMSysAvail_enum_ovrdflg
      link override Signal_Override/_ovrdval: Value=KOUTP_HVTHCMSysAvail_enum_ovrdval
  VACC_LVBattVoltSta_enum_Inproc : FVT_lib/outp/OverrideAndLimit  SystemSampleTime=-1  VariantActivationTime=update diagram  Latency=0  AutoFrameSizeCalculation=off
      link override Signal_Limit/_maxval: Value=KOUTP_LVBattVoltSta_enum_maxval
      link override Signal_Limit/_minval: Value=KOUTP_LVBattVoltSta_enum_minval
      link override Signal_Override/_ovrdflg: Value=KOUTP_LVBattVoltSta_enum_ovrdflg
      link override Signal_Override/_ovrdval: Value=KOUTP_LVBattVoltSta_enum_ovrdval
  VACC_VehHVPwrAvail4THCM_W_Inproc : FVT_lib/outp/OverrideAndLimit  SystemSampleTime=-1  VariantActivationTime=update diagram  Latency=0  AutoFrameSizeCalculation=off
      link override Signal_Limit/_maxval: Value=KOUTP_VehHVPwrAvail4THCM_W_maxval
      link override Signal_Limit/_minval: Value=KOUTP_VehHVPwrAvail4THCM_W_minval
      link override Signal_Override/_ovrdflg: Value=KOUTP_VehHVPwrAvail4THCM_W_ovrdflg
      link override Signal_Override/_ovrdval: Value=KOUTP_VehHVPwrAvail4THCM_W_ovrdval
  VAPM_ABSActiveTimeOut_flg_Inproc : FVT_lib/outp/OverrideAndLimit  SystemSampleTime=-1  VariantActivationTime=update diagram  Latency=0  AutoFrameSizeCalculation=off
      link override Signal_Limit/_maxval: Value=KOUTP_ABSActiveTimeOut_flg_maxval
      link override Signal_Limit/_minval: Value=KOUTP_ABSActiveTimeOut_flg_minval
      link override Signal_Override/_ovrdflg: Value=KOUTP_ABSActiveTimeOut_flg_ovrdflg
      link override Signal_Override/_ovrdval: Value=KOUTP_ABSActiveTimeOut_flg_ovrdval
  VAPM_ABSActiveToAPM_flg_Inproc : FVT_lib/outp/OverrideAndLimit  SystemSampleTime=-1  VariantActivationTime=update diagram  Latency=0  AutoFrameSizeCalculation=off
      link override Signal_Limit/_maxval: Value=KOUTP_ABSActiveToAPM_flg_maxval
      link override Signal_Limit/_minval: Value=KOUTP_ABSActiveToAPM_flg_minval
      link override Signal_Override/_ovrdflg: Value=KOUTP_ABSActiveToAPM_flg_ovrdflg
      link override Signal_Override/_ovrdval: Value=KOUTP_ABSActiveToAPM_flg_ovrdval
  VAPM_APSAngleTarget_Deg_Inproc : FVT_lib/outp/OverrideAndLimit  SystemSampleTime=-1  VariantActivationTime=update diagram  Latency=0  AutoFrameSizeCalculation=off
      link override Signal_Limit/_maxval: Value=KOUTP_APSAngleTarget_Deg_maxval
      link override Signal_Limit/_minval: Value=KOUTP_APSAngleTarget_Deg_minval
      link override Signal_Override/_ovrdflg: Value=KOUTP_APSAngleTarget_Deg_ovrdflg
      link override Signal_Override/_ovrdval: Value=KOUTP_APSAngleTarget_Deg_ovrdval
  VAPM_APSDFLL_cm_Inproc : FVT_lib/outp/OverrideAndLimit  SystemSampleTime=-1  VariantActivationTime=update diagram  Latency=0  AutoFrameSizeCalculation=off
      link override Signal_Limit/_maxval: Value=KOUTP_APSDFLL_cm_maxval
      link override Signal_Limit/_minval: Value=KOUTP_APSDFLL_cm_minval
      link override Signal_Override/_ovrdflg: Value=KOUTP_APSDFLL_cm_ovrdflg
      link override Signal_Override/_ovrdval: Value=KOUTP_APSDFLL_cm_ovrdval
  VAPM_APSDFLR_cm_Inproc : FVT_lib/outp/OverrideAndLimit  SystemSampleTime=-1  VariantActivationTime=update diagram  Latency=0  AutoFrameSizeCalculation=off
      link override Signal_Limit/_maxval: Value=KOUTP_APSDFLR_cm_maxval
      link override Signal_Limit/_minval: Value=KOUTP_APSDFLR_cm_minval
      link override Signal_Override/_ovrdflg: Value=KOUTP_APSDFLR_cm_ovrdflg
      link override Signal_Override/_ovrdval: Value=KOUTP_APSDFLR_cm_ovrdval
  VAPM_APSDRLL_cm_Inproc : FVT_lib/outp/OverrideAndLimit  SystemSampleTime=-1  VariantActivationTime=update diagram  Latency=0  AutoFrameSizeCalculation=off
      link override Signal_Limit/_maxval: Value=KOUTP_APSDRLL_cm_maxval
      link override Signal_Limit/_minval: Value=KOUTP_APSDRLL_cm_minval
      link override Signal_Override/_ovrdflg: Value=KOUTP_APSDRLL_cm_ovrdflg
      link override Signal_Override/_ovrdval: Value=KOUTP_APSDRLL_cm_ovrdval
  VAPM_APSDRLR_cm_Inproc : FVT_lib/outp/OverrideAndLimit  SystemSampleTime=-1  VariantActivationTime=update diagram  Latency=0  AutoFrameSizeCalculation=off
      link override Signal_Limit/_maxval: Value=KOUTP_APSDRLR_cm_maxval
      link override Signal_Limit/_minval: Value=KOUTP_APSDRLR_cm_minval
      link override Signal_Override/_ovrdflg: Value=KOUTP_APSDRLR_cm_ovrdflg
      link override Signal_Override/_ovrdval: Value=KOUTP_APSDRLR_cm_ovrdval
  VAPM_APSExitCondition_enum_Inproc : FVT_lib/outp/OverrideAndLimit  SystemSampleTime=-1  VariantActivationTime=update diagram  Latency=0  AutoFrameSizeCalculation=off
      link override Signal_Limit/_maxval: Value=KOUTP_APSExitCondition_enum_maxval
      link override Signal_Limit/_minval: Value=KOUTP_APSExitCondition_enum_minval
      link override Signal_Override/_ovrdflg: Value=KOUTP_APSExitCondition_enum_ovrdflg
      link override Signal_Override/_ovrdval: Value=KOUTP_APSExitCondition_enum_ovrdval
  VAPM_APSHWVer_enum_Inproc : FVT_lib/outp/OverrideAndLimit  SystemSampleTime=-1  VariantActivationTime=update diagram  Latency=0  AutoFrameSizeCalculation=off
      link override Signal_Limit/_maxval: Value=KOUTP_APSHWVer_enum_maxval
      link override Signal_Limit/_minval: Value=KOUTP_APSHWVer_enum_minval
      link override Signal_Override/_ovrdflg: Value=KOUTP_APSHWVer_enum_ovrdflg
      link override Signal_Override/_ovrdval: Value=KOUTP_APSHWVer_enum_ovrdval
  VAPM_APSProgressPCT_pct_Inproc : FVT_lib/outp/OverrideAndLimit  SystemSampleTime=-1  VariantActivationTime=update diagram  Latency=0  AutoFrameSizeCalculation=off
      link override Signal_Limit/_maxval: Value=KOUTP_APSProgressPCT_pct_maxval
      link override Signal_Limit/_minval: Value=KOUTP_APSProgressPCT_pct_minval
      link override Signal_Override/_ovrdflg: Value=KOUTP_APSProgressPCT_pct_ovrdflg
      link override Signal_Override/_ovrdval: Value=KOUTP_APSProgressPCT_pct_ovrdval
  VAPM_APSRQDisplay_enum_Inproc : FVT_lib/outp/OverrideAndLimit  SystemSampleTime=-1  VariantActivationTime=update diagram  Latency=0  AutoFrameSizeCalculation=off
      link override Signal_Limit/_maxval: Value=KOUTP_APSRQDisplay_enum_maxval
      link override Signal_Limit/_minval: Value=KOUTP_APSRQDisplay_enum_minval
      link override Signal_Override/_ovrdflg: Value=KOUTP_APSRQDisplay_enum_ovrdflg
      link override Signal_Override/_ovrdval: Value=KOUTP_APSRQDisplay_enum_ovrdval
  VAPM_APSRqEPASCtrl_flg_Inproc : FVT_lib/outp/OverrideAndLimit  SystemSampleTime=-1  VariantActivationTime=update diagram  Latency=0  AutoFrameSizeCalculation=off
      link override Signal_Limit/_maxval: Value=KOUTP_APSRqEPASCtrl_flg_maxval
      link override Signal_Limit/_minval: Value=KOUTP_APSRqEPASCtrl_flg_minval
      link override Signal_Override/_ovrdflg: Value=KOUTP_APSRqEPASCtrl_flg_ovrdflg
      link override Signal_Override/_ovrdval: Value=KOUTP_APSRqEPASCtrl_flg_ovrdval
  VAPM_APSSWVer_enum_Inproc : FVT_lib/outp/OverrideAndLimit  SystemSampleTime=-1  VariantActivationTime=update diagram  Latency=0  AutoFrameSizeCalculation=off
      link override Signal_Limit/_maxval: Value=KOUTP_APSSWVer_enum_maxval
      link override Signal_Limit/_minval: Value=KOUTP_APSSWVer_enum_minval
      link override Signal_Override/_ovrdflg: Value=KOUTP_APSSWVer_enum_ovrdflg
      link override Signal_Override/_ovrdval: Value=KOUTP_APSSWVer_enum_ovrdval
  VAPM_APSVRqEPASCtrl_flg_Inproc : FVT_lib/outp/OverrideAndLimit  SystemSampleTime=-1  VariantActivationTime=update diagram  Latency=0  AutoFrameSizeCalculation=off
      link override Signal_Limit/_maxval: Value=KOUTP_APSVRqEPASCtrl_flg_maxval
      link override Signal_Limit/_minval: Value=KOUTP_APSVRqEPASCtrl_flg_minval
      link override Signal_Override/_ovrdflg: Value=KOUTP_APSVRqEPASCtrl_flg_ovrdflg
      link override Signal_Override/_ovrdval: Value=KOUTP_APSVRqEPASCtrl_flg_ovrdval
  VAPM_AVMErrSTATimeOut_flg_Inproc : FVT_lib/outp/OverrideAndLimit  SystemSampleTime=-1  VariantActivationTime=update diagram  Latency=0  AutoFrameSizeCalculation=off
      link override Signal_Limit/_maxval: Value=KOUTP_AVMErrSTATimeOut_flg_maxval
      link override Signal_Limit/_minval: Value=KOUTP_AVMErrSTATimeOut_flg_minval
      link override Signal_Override/_ovrdflg: Value=KOUTP_AVMErrSTATimeOut_flg_ovrdflg
      link override Signal_Override/_ovrdval: Value=KOUTP_AVMErrSTATimeOut_flg_ovrdval
  VAPM_AVMErrSTA_flg_Inproc : FVT_lib/outp/OverrideAndLimit  SystemSampleTime=-1  VariantActivationTime=update diagram  Latency=0  AutoFrameSizeCalculation=off
      link override Signal_Limit/_maxval: Value=KOUTP_AVMErrSTA_flg_maxval
      link override Signal_Limit/_minval: Value=KOUTP_AVMErrSTA_flg_minval
      link override Signal_Override/_ovrdflg: Value=KOUTP_AVMErrSTA_flg_ovrdflg
      link override Signal_Override/_ovrdval: Value=KOUTP_AVMErrSTA_flg_ovrdval
  VAPM_AVMParkingmodeTimeOut_flg_Inproc : FVT_lib/outp/OverrideAndLimit  SystemSampleTime=-1  VariantActivationTime=update diagram  Latency=0  AutoFrameSizeCalculation=off
      link override Signal_Limit/_maxval: Value=KOUTP_AVMParkingmodeTimeOut_flg_maxval
      link override Signal_Limit/_minval: Value=KOUTP_AVMParkingmodeTimeOut_flg_minval
      link override Signal_Override/_ovrdflg: Value=KOUTP_AVMParkingmodeTimeOut_flg_ovrdflg
      link override Signal_Override/_ovrdval: Value=KOUTP_AVMParkingmodeTimeOut_flg_ovrdval
  VAPM_AVMParkingmode_enum_Inproc : FVT_lib/outp/OverrideAndLimit  SystemSampleTime=-1  VariantActivationTime=update diagram  Latency=0  AutoFrameSizeCalculation=off
      link override Signal_Limit/_maxval: Value=KOUTP_AVMParkingmode_enum_maxval
      link override Signal_Limit/_minval: Value=KOUTP_AVMParkingmode_enum_minval
      link override Signal_Override/_ovrdflg: Value=KOUTP_AVMParkingmode_enum_ovrdflg
      link override Signal_Override/_ovrdval: Value=KOUTP_AVMParkingmode_enum_ovrdval
  VAPM_AVMparkingcancelTimeOut_flg_Inproc : FVT_lib/outp/OverrideAndLimit  SystemSampleTime=-1  VariantActivationTime=update diagram  Latency=0  AutoFrameSizeCalculation=off
      link override Signal_Limit/_maxval: Value=KOUTP_AVMparkingcancelTimeOut_flg_maxval
      link override Signal_Limit/_minval: Value=KOUTP_AVMparkingcancelTimeOut_flg_minval
      link override Signal_Override/_ovrdflg: Value=KOUTP_AVMparkingcancelTimeOut_flg_ovrdflg
      link override Signal_Override/_ovrdval: Value=KOUTP_AVMparkingcancelTimeOut_flg_ovrdval
  VAPM_AVMparkingcancel_enum_Inproc : FVT_lib/outp/OverrideAndLimit  SystemSampleTime=-1  VariantActivationTime=update diagram  Latency=0  AutoFrameSizeCalculation=off
      link override Signal_Limit/_maxval: Value=KOUTP_AVMparkingcancel_enum_maxval
      link override Signal_Limit/_minval: Value=KOUTP_AVMparkingcancel_enum_minval
      link override Signal_Override/_ovrdflg: Value=KOUTP_AVMparkingcancel_enum_ovrdflg
      link override Signal_Override/_ovrdval: Value=KOUTP_AVMparkingcancel_enum_ovrdval
  VAPM_AVMparkingexcuteTimeOut_flg_Inproc : FVT_lib/outp/OverrideAndLimit  SystemSampleTime=-1  VariantActivationTime=update diagram  Latency=0  AutoFrameSizeCalculation=off
      link override Signal_Limit/_maxval: Value=KOUTP_AVMparkingexcuteTimeOut_flg_maxval
      link override Signal_Limit/_minval: Value=KOUTP_AVMparkingexcuteTimeOut_flg_minval
      link override Signal_Override/_ovrdflg: Value=KOUTP_AVMparkingexcuteTimeOut_flg_ovrdflg
      link override Signal_Override/_ovrdval: Value=KOUTP_AVMparkingexcuteTimeOut_flg_ovrdval
  VAPM_AVMparkingexcute_enum_Inproc : FVT_lib/outp/OverrideAndLimit  SystemSampleTime=-1  VariantActivationTime=update diagram  Latency=0  AutoFrameSizeCalculation=off
      link override Signal_Limit/_maxval: Value=KOUTP_AVMparkingexcute_enum_maxval
      link override Signal_Limit/_minval: Value=KOUTP_AVMparkingexcute_enum_minval
      link override Signal_Override/_ovrdflg: Value=KOUTP_AVMparkingexcute_enum_ovrdflg
      link override Signal_Override/_ovrdval: Value=KOUTP_AVMparkingexcute_enum_ovrdval
  VAPM_BrkPedalPosTimeOut_flg_Inproc : FVT_lib/outp/OverrideAndLimit  SystemSampleTime=-1  VariantActivationTime=update diagram  Latency=0  AutoFrameSizeCalculation=off
      link override Signal_Limit/_maxval: Value=KOUTP_BrkPedalPosTimeOut_flg_maxval
      link override Signal_Limit/_minval: Value=KOUTP_BrkPedalPosTimeOut_flg_minval
      link override Signal_Override/_ovrdflg: Value=KOUTP_BrkPedalPosTimeOut_flg_ovrdflg
      link override Signal_Override/_ovrdval: Value=KOUTP_BrkPedalPosTimeOut_flg_ovrdval
  VAPM_BrkPedalPosToAPM_pct_Inproc : FVT_lib/outp/OverrideAndLimit  SystemSampleTime=-1  VariantActivationTime=update diagram  Latency=0  AutoFrameSizeCalculation=off
      link override Signal_Limit/_maxval: Value=KOUTP_BrkPedalPosToAPM_pct_maxval
      link override Signal_Limit/_minval: Value=KOUTP_BrkPedalPosToAPM_pct_minval
      link override Signal_Override/_ovrdflg: Value=KOUTP_BrkPedalPosToAPM_pct_ovrdflg
      link override Signal_Override/_ovrdval: Value=KOUTP_BrkPedalPosToAPM_pct_ovrdval
  VAPM_BrkSwStaTimeOut_flg_Inproc : FVT_lib/outp/OverrideAndLimit  SystemSampleTime=-1  VariantActivationTime=update diagram  Latency=0  AutoFrameSizeCalculation=off
      link override Signal_Limit/_maxval: Value=KOUTP_BrkSwStaTimeOut_flg_maxval
      link override Signal_Limit/_minval: Value=KOUTP_BrkSwStaTimeOut_flg_minval
      link override Signal_Override/_ovrdflg: Value=KOUTP_BrkSwStaTimeOut_flg_ovrdflg
      link override Signal_Override/_ovrdval: Value=KOUTP_BrkSwStaTimeOut_flg_ovrdval
  VAPM_BrkSwSta_flg_Inproc : FVT_lib/outp/OverrideAndLimit  SystemSampleTime=-1  VariantActivationTime=update diagram  Latency=0  AutoFrameSizeCalculation=off
      link override Signal_Limit/_maxval: Value=KOUTP_BrkSwSta_flg_maxval
      link override Signal_Limit/_minval: Value=KOUTP_BrkSwSta_flg_minval
      link override Signal_Override/_ovrdflg: Value=KOUTP_BrkSwSta_flg_ovrdflg
      link override Signal_Override/_ovrdval: Value=KOUTP_BrkSwSta_flg_ovrdval
  VAPM_BrkSwVTimeOut_flg_Inproc : FVT_lib/outp/OverrideAndLimit  SystemSampleTime=-1  VariantActivationTime=update diagram  Latency=0  AutoFrameSizeCalculation=off
      link override Signal_Limit/_maxval: Value=KOUTP_BrkSwVTimeOut_flg_maxval
      link override Signal_Limit/_minval: Value=KOUTP_BrkSwVTimeOut_flg_minval
      link override Signal_Override/_ovrdflg: Value=KOUTP_BrkSwVTimeOut_flg_ovrdflg
      link override Signal_Override/_ovrdval: Value=KOUTP_BrkSwVTimeOut_flg_ovrdval
  VAPM_BrkSwV_flg_Inproc : FVT_lib/outp/OverrideAndLimit  SystemSampleTime=-1  VariantActivationTime=update diagram  Latency=0  AutoFrameSizeCalculation=off
      link override Signal_Limit/_maxval: Value=KOUTP_BrkSwV_flg_maxval
      link override Signal_Limit/_minval: Value=KOUTP_BrkSwV_flg_minval
      link override Signal_Override/_ovrdflg: Value=KOUTP_BrkSwV_flg_ovrdflg
      link override Signal_Override/_ovrdval: Value=KOUTP_BrkSwV_flg_ovrdval
  VAPM_CAASSta_enum_Inproc : FVT_lib/outp/OverrideAndLimit  SystemSampleTime=-1  VariantActivationTime=update diagram  Latency=0  AutoFrameSizeCalculation=off
      link override Signal_Limit/_maxval: Value=KOUTP_CAASSta_enum_maxval
      link override Signal_Limit/_minval: Value=KOUTP_CAASSta_enum_minval
      link override Signal_Override/_ovrdflg: Value=KOUTP_CAASSta_enum_ovrdflg
      link override Signal_Override/_ovrdval: Value=KOUTP_CAASSta_enum_ovrdval
  VAPM_CAASSwTimeOut_flg_Inproc : FVT_lib/outp/OverrideAndLimit  SystemSampleTime=-1  VariantActivationTime=update diagram  Latency=0  AutoFrameSizeCalculation=off
      link override Signal_Limit/_maxval: Value=KOUTP_CAASSwTimeOut_flg_maxval
      link override Signal_Limit/_minval: Value=KOUTP_CAASSwTimeOut_flg_minval
      link override Signal_Override/_ovrdflg: Value=KOUTP_CAASSwTimeOut_flg_ovrdflg
      link override Signal_Override/_ovrdval: Value=KOUTP_CAASSwTimeOut_flg_ovrdval
  VAPM_CAASSw_enum_Inproc : FVT_lib/outp/OverrideAndLimit  SystemSampleTime=-1  VariantActivationTime=update diagram  Latency=0  AutoFrameSizeCalculation=off
      link override Signal_Limit/_maxval: Value=KOUTP_CAASSw_enum_maxval
      link override Signal_Limit/_minval: Value=KOUTP_CAASSw_enum_minval
      link override Signal_Override/_ovrdflg: Value=KOUTP_CAASSw_enum_ovrdflg
      link override Signal_Override/_ovrdval: Value=KOUTP_CAASSw_enum_ovrdval
  VAPM_Chime_enum_Inproc : FVT_lib/outp/OverrideAndLimit  SystemSampleTime=-1  VariantActivationTime=update diagram  Latency=0  AutoFrameSizeCalculation=off
      link override Signal_Limit/_maxval: Value=KOUTP_Chime_enum_maxval
      link override Signal_Limit/_minval: Value=KOUTP_Chime_enum_minval
      link override Signal_Override/_ovrdflg: Value=KOUTP_Chime_enum_ovrdflg
      link override Signal_Override/_ovrdval: Value=KOUTP_Chime_enum_ovrdval
  VAPM_ChrgPlugSta_enum_Inproc : FVT_lib/outp/OverrideAndLimit  SystemSampleTime=-1  VariantActivationTime=update diagram  Latency=0  AutoFrameSizeCalculation=off
      link override Signal_Limit/_maxval: Value=KOUTP_ChrgPlugSta_enum_maxval
      link override Signal_Limit/_minval: Value=KOUTP_ChrgPlugSta_enum_minval
      link override Signal_Override/_ovrdflg: Value=KOUTP_ChrgPlugSta_enum_ovrdflg
      link override Signal_Override/_ovrdval: Value=KOUTP_ChrgPlugSta_enum_ovrdval
  VAPM_DriIntendTimeOut_flg_Inproc : FVT_lib/outp/OverrideAndLimit  SystemSampleTime=-1  VariantActivationTime=update diagram  Latency=0  AutoFrameSizeCalculation=off
      link override Signal_Limit/_maxval: Value=KOUTP_DriIntendTimeOut_flg_maxval
      link override Signal_Limit/_minval: Value=KOUTP_DriIntendTimeOut_flg_minval
      link override Signal_Override/_ovrdflg: Value=KOUTP_DriIntendTimeOut_flg_ovrdflg
      link override Signal_Override/_ovrdval: Value=KOUTP_DriIntendTimeOut_flg_ovrdval
  VAPM_DriIntend_enum_Inproc : FVT_lib/outp/OverrideAndLimit  SystemSampleTime=-1  VariantActivationTime=update diagram  Latency=0  AutoFrameSizeCalculation=off
      link override Signal_Limit/_maxval: Value=KOUTP_DriIntend_enum_maxval
      link override Signal_Limit/_minval: Value=KOUTP_DriIntend_enum_minval
      link override Signal_Override/_ovrdflg: Value=KOUTP_DriIntend_enum_ovrdflg
      link override Signal_Override/_ovrdval: Value=KOUTP_DriIntend_enum_ovrdval
  VAPM_DriverSeatBeltCmdTimeOut_flg_Inproc : FVT_lib/outp/OverrideAndLimit  SystemSampleTime=-1  VariantActivationTime=update diagram  Latency=0  AutoFrameSizeCalculation=off
      link override Signal_Limit/_maxval: Value=KOUTP_DriverSeatBeltCmdTimeOut_flg_maxval
      link override Signal_Limit/_minval: Value=KOUTP_DriverSeatBeltCmdTimeOut_flg_minval
      link override Signal_Override/_ovrdflg: Value=KOUTP_DriverSeatBeltCmdTimeOut_flg_ovrdflg
      link override Signal_Override/_ovrdval: Value=KOUTP_DriverSeatBeltCmdTimeOut_flg_ovrdval
  VAPM_DriverSeatBeltCmd_flg_Inproc : FVT_lib/outp/OverrideAndLimit  SystemSampleTime=-1  VariantActivationTime=update diagram  Latency=0  AutoFrameSizeCalculation=off
      link override Signal_Limit/_maxval: Value=KOUTP_DriverSeatBeltCmd_flg_maxval
      link override Signal_Limit/_minval: Value=KOUTP_DriverSeatBeltCmd_flg_minval
      link override Signal_Override/_ovrdflg: Value=KOUTP_DriverSeatBeltCmd_flg_ovrdflg
      link override Signal_Override/_ovrdval: Value=KOUTP_DriverSeatBeltCmd_flg_ovrdval
  VAPM_EPBErrStaTimeOut_flg_Inproc : FVT_lib/outp/OverrideAndLimit  SystemSampleTime=-1  VariantActivationTime=update diagram  Latency=0  AutoFrameSizeCalculation=off
      link override Signal_Limit/_maxval: Value=KOUTP_EPBErrStaTimeOut_flg_maxval
      link override Signal_Limit/_minval: Value=KOUTP_EPBErrStaTimeOut_flg_minval
      link override Signal_Override/_ovrdflg: Value=KOUTP_EPBErrStaTimeOut_flg_ovrdflg
      link override Signal_Override/_ovrdval: Value=KOUTP_EPBErrStaTimeOut_flg_ovrdval
  VAPM_EPBErrSta_enum_Inproc : FVT_lib/outp/OverrideAndLimit  SystemSampleTime=-1  VariantActivationTime=update diagram  Latency=0  AutoFrameSizeCalculation=off
      link override Signal_Limit/_maxval: Value=KOUTP_EPBErrSta_enum_maxval
      link override Signal_Limit/_minval: Value=KOUTP_EPBErrSta_enum_minval
      link override Signal_Override/_ovrdflg: Value=KOUTP_EPBErrSta_enum_ovrdflg
      link override Signal_Override/_ovrdval: Value=KOUTP_EPBErrSta_enum_ovrdval
  VAPM_EPBExtApplyAvailTimeOut_flg_Inproc : FVT_lib/outp/OverrideAndLimit  SystemSampleTime=-1  VariantActivationTime=update diagram  Latency=0  AutoFrameSizeCalculation=off
      link override Signal_Limit/_maxval: Value=KOUTP_EPBExtApplyAvailTimeOut_flg_maxval
      link override Signal_Limit/_minval: Value=KOUTP_EPBExtApplyAvailTimeOut_flg_minval
      link override Signal_Override/_ovrdflg: Value=KOUTP_EPBExtApplyAvailTimeOut_flg_ovrdflg
      link override Signal_Override/_ovrdval: Value=KOUTP_EPBExtApplyAvailTimeOut_flg_ovrdval
  VAPM_EPBExtApplyAvail_flg_Inproc : FVT_lib/outp/OverrideAndLimit  SystemSampleTime=-1  VariantActivationTime=update diagram  Latency=0  AutoFrameSizeCalculation=off
      link override Signal_Limit/_maxval: Value=KOUTP_EPBExtApplyAvail_flg_maxval
      link override Signal_Limit/_minval: Value=KOUTP_EPBExtApplyAvail_flg_minval
      link override Signal_Override/_ovrdflg: Value=KOUTP_EPBExtApplyAvail_flg_ovrdflg
      link override Signal_Override/_ovrdval: Value=KOUTP_EPBExtApplyAvail_flg_ovrdval
  VAPM_EPBExtReleaseAvailTimeOut_flg_Inproc : FVT_lib/outp/OverrideAndLimit  SystemSampleTime=-1  VariantActivationTime=update diagram  Latency=0  AutoFrameSizeCalculation=off
      link override Signal_Limit/_maxval: Value=KOUTP_EPBExtReleaseAvailTimeOut_flg_maxval
      link override Signal_Limit/_minval: Value=KOUTP_EPBExtReleaseAvailTimeOut_flg_minval
      link override Signal_Override/_ovrdflg: Value=KOUTP_EPBExtReleaseAvailTimeOut_flg_ovrdflg
      link override Signal_Override/_ovrdval: Value=KOUTP_EPBExtReleaseAvailTimeOut_flg_ovrdval
  VAPM_EPBExtReleaseAvail_flg_Inproc : FVT_lib/outp/OverrideAndLimit  SystemSampleTime=-1  VariantActivationTime=update diagram  Latency=0  AutoFrameSizeCalculation=off
      link override Signal_Limit/_maxval: Value=KOUTP_EPBExtReleaseAvail_flg_maxval
      link override Signal_Limit/_minval: Value=KOUTP_EPBExtReleaseAvail_flg_minval
      link override Signal_Override/_ovrdflg: Value=KOUTP_EPBExtReleaseAvail_flg_ovrdflg
      link override Signal_Override/_ovrdval: Value=KOUTP_EPBExtReleaseAvail_flg_ovrdval
  VAPM_EPBStaTimeOut_flg_Inproc : FVT_lib/outp/OverrideAndLimit  SystemSampleTime=-1  VariantActivationTime=update diagram  Latency=0  AutoFrameSizeCalculation=off
      link override Signal_Limit/_maxval: Value=KOUTP_EPBStaTimeOut_flg_maxval
      link override Signal_Limit/_minval: Value=KOUTP_EPBStaTimeOut_flg_minval
      link override Signal_Override/_ovrdflg: Value=KOUTP_EPBStaTimeOut_flg_ovrdflg
      link override Signal_Override/_ovrdval: Value=KOUTP_EPBStaTimeOut_flg_ovrdval
  VAPM_EPBSta_enum_Inproc : FVT_lib/outp/OverrideAndLimit  SystemSampleTime=-1  VariantActivationTime=update diagram  Latency=0  AutoFrameSizeCalculation=off
      link override Signal_Limit/_maxval: Value=KOUTP_EPBSta_enum_maxval
      link override Signal_Limit/_minval: Value=KOUTP_EPBSta_enum_minval
      link override Signal_Override/_ovrdflg: Value=KOUTP_EPBSta_enum_ovrdflg
      link override Signal_Override/_ovrdval: Value=KOUTP_EPBSta_enum_ovrdval
  VAPM_EPSAOIControlTimeOut_flg_Inproc : FVT_lib/outp/OverrideAndLimit  SystemSampleTime=-1  VariantActivationTime=update diagram  Latency=0  AutoFrameSizeCalculation=off
      link override Signal_Limit/_maxval: Value=KOUTP_EPSAOIControlTimeOut_flg_maxval
      link override Signal_Limit/_minval: Value=KOUTP_EPSAOIControlTimeOut_flg_minval
      link override Signal_Override/_ovrdflg: Value=KOUTP_EPSAOIControlTimeOut_flg_ovrdflg
      link override Signal_Override/_ovrdval: Value=KOUTP_EPSAOIControlTimeOut_flg_ovrdval
  VAPM_EPSAOIControl_enum_Inproc : FVT_lib/outp/OverrideAndLimit  SystemSampleTime=-1  VariantActivationTime=update diagram  Latency=0  AutoFrameSizeCalculation=off
      link override Signal_Limit/_maxval: Value=KOUTP_EPSAOIControl_enum_maxval
      link override Signal_Limit/_minval: Value=KOUTP_EPSAOIControl_enum_minval
      link override Signal_Override/_ovrdflg: Value=KOUTP_EPSAOIControl_enum_ovrdflg
      link override Signal_Override/_ovrdval: Value=KOUTP_EPSAOIControl_enum_ovrdval
  VAPM_ESCAPSStaTimeOut_flg_Inproc : FVT_lib/outp/OverrideAndLimit  SystemSampleTime=-1  VariantActivationTime=update diagram  Latency=0  AutoFrameSizeCalculation=off
      link override Signal_Limit/_maxval: Value=KOUTP_ESCAPSStaTimeOut_flg_maxval
      link override Signal_Limit/_minval: Value=KOUTP_ESCAPSStaTimeOut_flg_minval
      link override Signal_Override/_ovrdflg: Value=KOUTP_ESCAPSStaTimeOut_flg_ovrdflg
      link override Signal_Override/_ovrdval: Value=KOUTP_ESCAPSStaTimeOut_flg_ovrdval
  VAPM_ESCAPSSta_enum_Inproc : FVT_lib/outp/OverrideAndLimit  SystemSampleTime=-1  VariantActivationTime=update diagram  Latency=0  AutoFrameSizeCalculation=off
      link override Signal_Limit/_maxval: Value=KOUTP_ESCAPSSta_enum_maxval
      link override Signal_Limit/_minval: Value=KOUTP_ESCAPSSta_enum_minval
      link override Signal_Override/_ovrdflg: Value=KOUTP_ESCAPSSta_enum_ovrdflg
      link override Signal_Override/_ovrdval: Value=KOUTP_ESCAPSSta_enum_ovrdval
  VAPM_ESCStandstillTimeOut_flg_Inproc : FVT_lib/outp/OverrideAndLimit  SystemSampleTime=-1  VariantActivationTime=update diagram  Latency=0  AutoFrameSizeCalculation=off
      link override Signal_Limit/_maxval: Value=KOUTP_ESCStandstillTimeOut_flg_maxval
      link override Signal_Limit/_minval: Value=KOUTP_ESCStandstillTimeOut_flg_minval
      link override Signal_Override/_ovrdflg: Value=KOUTP_ESCStandstillTimeOut_flg_ovrdflg
      link override Signal_Override/_ovrdval: Value=KOUTP_ESCStandstillTimeOut_flg_ovrdval
  VAPM_ESCStandstill_flg_Inproc : FVT_lib/outp/OverrideAndLimit  SystemSampleTime=-1  VariantActivationTime=update diagram  Latency=0  AutoFrameSizeCalculation=off
      link override Signal_Limit/_maxval: Value=KOUTP_ESCStandstill_flg_maxval
      link override Signal_Limit/_minval: Value=KOUTP_ESCStandstill_flg_minval
      link override Signal_Override/_ovrdflg: Value=KOUTP_ESCStandstill_flg_ovrdflg
      link override Signal_Override/_ovrdval: Value=KOUTP_ESCStandstill_flg_ovrdval
  VAPM_FSOffSwTimeOut_flg_Inproc : FVT_lib/outp/OverrideAndLimit  SystemSampleTime=-1  VariantActivationTime=update diagram  Latency=0  AutoFrameSizeCalculation=off
      link override Signal_Limit/_maxval: Value=KOUTP_FSOffSwTimeOut_flg_maxval
      link override Signal_Limit/_minval: Value=KOUTP_FSOffSwTimeOut_flg_minval
      link override Signal_Override/_ovrdflg: Value=KOUTP_FSOffSwTimeOut_flg_ovrdflg
      link override Signal_Override/_ovrdval: Value=KOUTP_FSOffSwTimeOut_flg_ovrdval
  VAPM_FSOffSw_enum_Inproc : FVT_lib/outp/OverrideAndLimit  SystemSampleTime=-1  VariantActivationTime=update diagram  Latency=0  AutoFrameSizeCalculation=off
      link override Signal_Limit/_maxval: Value=KOUTP_FSOffSw_enum_maxval
      link override Signal_Limit/_minval: Value=KOUTP_FSOffSw_enum_minval
      link override Signal_Override/_ovrdflg: Value=KOUTP_FSOffSw_enum_ovrdflg
      link override Signal_Override/_ovrdval: Value=KOUTP_FSOffSw_enum_ovrdval
  VAPM_GRADETimeOut_flg_Inproc : FVT_lib/outp/OverrideAndLimit  SystemSampleTime=-1  VariantActivationTime=update diagram  Latency=0  AutoFrameSizeCalculation=off
      link override Signal_Limit/_maxval: Value=KOUTP_GRADETimeOut_flg_maxval
      link override Signal_Limit/_minval: Value=KOUTP_GRADETimeOut_flg_minval
      link override Signal_Override/_ovrdflg: Value=KOUTP_GRADETimeOut_flg_ovrdflg
      link override Signal_Override/_ovrdval: Value=KOUTP_GRADETimeOut_flg_ovrdval
  VAPM_GRADE_Deg_Inproc : FVT_lib/outp/OverrideAndLimit  SystemSampleTime=-1  VariantActivationTime=update diagram  Latency=0  AutoFrameSizeCalculation=off
      link override Signal_Limit/_maxval: Value=KOUTP_GRADE_Deg_maxval
      link override Signal_Limit/_minval: Value=KOUTP_GRADE_Deg_minval
      link override Signal_Override/_ovrdflg: Value=KOUTP_GRADE_Deg_ovrdflg
      link override Signal_Override/_ovrdval: Value=KOUTP_GRADE_Deg_ovrdval
  VAPM_IVIScreenTimeOut_flg_Inproc : FVT_lib/outp/OverrideAndLimit  SystemSampleTime=-1  VariantActivationTime=update diagram  Latency=0  AutoFrameSizeCalculation=off
      link override Signal_Limit/_maxval: Value=KOUTP_IVIScreenTimeOut_flg_maxval
      link override Signal_Limit/_minval: Value=KOUTP_IVIScreenTimeOut_flg_minval
      link override Signal_Override/_ovrdflg: Value=KOUTP_IVIScreenTimeOut_flg_ovrdflg
      link override Signal_Override/_ovrdval: Value=KOUTP_IVIScreenTimeOut_flg_ovrdval
  VAPM_IVIScreen_enum_Inproc : FVT_lib/outp/OverrideAndLimit  SystemSampleTime=-1  VariantActivationTime=update diagram  Latency=0  AutoFrameSizeCalculation=off
      link override Signal_Limit/_maxval: Value=KOUTP_IVIScreen_enum_maxval
      link override Signal_Limit/_minval: Value=KOUTP_IVIScreen_enum_minval
      link override Signal_Override/_ovrdflg: Value=KOUTP_IVIScreen_enum_ovrdflg
      link override Signal_Override/_ovrdval: Value=KOUTP_IVIScreen_enum_ovrdval
  VAPM_IVIStatusTimeOut_flg_Inproc : FVT_lib/outp/OverrideAndLimit  SystemSampleTime=-1  VariantActivationTime=update diagram  Latency=0  AutoFrameSizeCalculation=off
      link override Signal_Limit/_maxval: Value=KOUTP_IVIStatusTimeOut_flg_maxval
      link override Signal_Limit/_minval: Value=KOUTP_IVIStatusTimeOut_flg_minval
      link override Signal_Override/_ovrdflg: Value=KOUTP_IVIStatusTimeOut_flg_ovrdflg
      link override Signal_Override/_ovrdval: Value=KOUTP_IVIStatusTimeOut_flg_ovrdval
  VAPM_IVIStatus_flg_Inproc : FVT_lib/outp/OverrideAndLimit  SystemSampleTime=-1  VariantActivationTime=update diagram  Latency=0  AutoFrameSizeCalculation=off
      link override Signal_Limit/_maxval: Value=KOUTP_IVIStatus_flg_maxval
      link override Signal_Limit/_minval: Value=KOUTP_IVIStatus_flg_minval
      link override Signal_Override/_ovrdflg: Value=KOUTP_IVIStatus_flg_ovrdflg
      link override Signal_Override/_ovrdval: Value=KOUTP_IVIStatus_flg_ovrdval
  VAPM_LFPulseCountTimeOut_flg_Inproc : FVT_lib/outp/OverrideAndLimit  SystemSampleTime=-1  VariantActivationTime=update diagram  Latency=0  AutoFrameSizeCalculation=off
      link override Signal_Limit/_maxval: Value=KOUTP_LFPulseCountTimeOut_flg_maxval
      link override Signal_Limit/_minval: Value=KOUTP_LFPulseCountTimeOut_flg_minval
      link override Signal_Override/_ovrdflg: Value=KOUTP_LFPulseCountTimeOut_flg_ovrdflg
      link override Signal_Override/_ovrdval: Value=KOUTP_LFPulseCountTimeOut_flg_ovrdval
  VAPM_LFPulseCountVTimeOut_flg_Inproc : FVT_lib/outp/OverrideAndLimit  SystemSampleTime=-1  VariantActivationTime=update diagram  Latency=0  AutoFrameSizeCalculation=off
      link override Signal_Limit/_maxval: Value=KOUTP_LFPulseCountVTimeOut_flg_maxval
      link override Signal_Limit/_minval: Value=KOUTP_LFPulseCountVTimeOut_flg_minval
      link override Signal_Override/_ovrdflg: Value=KOUTP_LFPulseCountVTimeOut_flg_ovrdflg
      link override Signal_Override/_ovrdval: Value=KOUTP_LFPulseCountVTimeOut_flg_ovrdval
  VAPM_LFPulseCountV_flg_Inproc : FVT_lib/outp/OverrideAndLimit  SystemSampleTime=-1  VariantActivationTime=update diagram  Latency=0  AutoFrameSizeCalculation=off
      link override Signal_Limit/_maxval: Value=KOUTP_LFPulseCountV_flg_maxval
      link override Signal_Limit/_minval: Value=KOUTP_LFPulseCountV_flg_minval
      link override Signal_Override/_ovrdflg: Value=KOUTP_LFPulseCountV_flg_ovrdflg
      link override Signal_Override/_ovrdval: Value=KOUTP_LFPulseCountV_flg_ovrdval
  VAPM_LFPulseCount_enum_Inproc : FVT_lib/outp/OverrideAndLimit  SystemSampleTime=-1  VariantActivationTime=update diagram  Latency=0  AutoFrameSizeCalculation=off
      link override Signal_Limit/_maxval: Value=KOUTP_LFPulseCount_enum_maxval
      link override Signal_Limit/_minval: Value=KOUTP_LFPulseCount_enum_minval
      link override Signal_Override/_ovrdflg: Value=KOUTP_LFPulseCount_enum_ovrdflg
      link override Signal_Override/_ovrdval: Value=KOUTP_LFPulseCount_enum_ovrdval
  VAPM_LFRawWhlSpeedTimeOut_flg_Inproc : FVT_lib/outp/OverrideAndLimit  SystemSampleTime=-1  VariantActivationTime=update diagram  Latency=0  AutoFrameSizeCalculation=off
      link override Signal_Limit/_maxval: Value=KOUTP_LFRawWhlSpeedTimeOut_flg_maxval
      link override Signal_Limit/_minval: Value=KOUTP_LFRawWhlSpeedTimeOut_flg_minval
      link override Signal_Override/_ovrdflg: Value=KOUTP_LFRawWhlSpeedTimeOut_flg_ovrdflg
      link override Signal_Override/_ovrdval: Value=KOUTP_LFRawWhlSpeedTimeOut_flg_ovrdval
  VAPM_LFRawWhlSpeedVTimeOut_flg_Inproc : FVT_lib/outp/OverrideAndLimit  SystemSampleTime=-1  VariantActivationTime=update diagram  Latency=0  AutoFrameSizeCalculation=off
      link override Signal_Limit/_maxval: Value=KOUTP_LFRawWhlSpeedVTimeOut_flg_maxval
      link override Signal_Limit/_minval: Value=KOUTP_LFRawWhlSpeedVTimeOut_flg_minval
      link override Signal_Override/_ovrdflg: Value=KOUTP_LFRawWhlSpeedVTimeOut_flg_ovrdflg
      link override Signal_Override/_ovrdval: Value=KOUTP_LFRawWhlSpeedVTimeOut_flg_ovrdval
  VAPM_LFRawWhlSpeedV_flg_Inproc : FVT_lib/outp/OverrideAndLimit  SystemSampleTime=-1  VariantActivationTime=update diagram  Latency=0  AutoFrameSizeCalculation=off
      link override Signal_Limit/_maxval: Value=KOUTP_LFRawWhlSpeedV_flg_maxval
      link override Signal_Limit/_minval: Value=KOUTP_LFRawWhlSpeedV_flg_minval
      link override Signal_Override/_ovrdflg: Value=KOUTP_LFRawWhlSpeedV_flg_ovrdflg
      link override Signal_Override/_ovrdval: Value=KOUTP_LFRawWhlSpeedV_flg_ovrdval
  VAPM_LFRawWhlSpeed_kph_Inproc : FVT_lib/outp/OverrideAndLimit  SystemSampleTime=-1  VariantActivationTime=update diagram  Latency=0  AutoFrameSizeCalculation=off
      link override Signal_Limit/_maxval: Value=KOUTP_LFRawWhlSpeed_kph_maxval
      link override Signal_Limit/_minval: Value=KOUTP_LFRawWhlSpeed_kph_minval
      link override Signal_Override/_ovrdflg: Value=KOUTP_LFRawWhlSpeed_kph_ovrdflg
      link override Signal_Override/_ovrdval: Value=KOUTP_LFRawWhlSpeed_kph_ovrdval
  VAPM_LFWhlRotDirTimeOut_flg_Inproc : FVT_lib/outp/OverrideAndLimit  SystemSampleTime=-1  VariantActivationTime=update diagram  Latency=0  AutoFrameSizeCalculation=off
      link override Signal_Limit/_maxval: Value=KOUTP_LFWhlRotDirTimeOut_flg_maxval
      link override Signal_Limit/_minval: Value=KOUTP_LFWhlRotDirTimeOut_flg_minval
      link override Signal_Override/_ovrdflg: Value=KOUTP_LFWhlRotDirTimeOut_flg_ovrdflg
      link override Signal_Override/_ovrdval: Value=KOUTP_LFWhlRotDirTimeOut_flg_ovrdval
  VAPM_LFWhlRotDir_enum_Inproc : FVT_lib/outp/OverrideAndLimit  SystemSampleTime=-1  VariantActivationTime=update diagram  Latency=0  AutoFrameSizeCalculation=off
      link override Signal_Limit/_maxval: Value=KOUTP_LFWhlRotDir_enum_maxval
      link override Signal_Limit/_minval: Value=KOUTP_LFWhlRotDir_enum_minval
      link override Signal_Override/_ovrdflg: Value=KOUTP_LFWhlRotDir_enum_ovrdflg
      link override Signal_Override/_ovrdval: Value=KOUTP_LFWhlRotDir_enum_ovrdval
  VAPM_LRPulseCountTimeOut_flg_Inproc : FVT_lib/outp/OverrideAndLimit  SystemSampleTime=-1  VariantActivationTime=update diagram  Latency=0  AutoFrameSizeCalculation=off
      link override Signal_Limit/_maxval: Value=KOUTP_LRPulseCountTimeOut_flg_maxval
      link override Signal_Limit/_minval: Value=KOUTP_LRPulseCountTimeOut_flg_minval
      link override Signal_Override/_ovrdflg: Value=KOUTP_LRPulseCountTimeOut_flg_ovrdflg
      link override Signal_Override/_ovrdval: Value=KOUTP_LRPulseCountTimeOut_flg_ovrdval
  VAPM_LRPulseCountVTimeOut_flg_Inproc : FVT_lib/outp/OverrideAndLimit  SystemSampleTime=-1  VariantActivationTime=update diagram  Latency=0  AutoFrameSizeCalculation=off
      link override Signal_Limit/_maxval: Value=KOUTP_LRPulseCountVTimeOut_flg_maxval
      link override Signal_Limit/_minval: Value=KOUTP_LRPulseCountVTimeOut_flg_minval
      link override Signal_Override/_ovrdflg: Value=KOUTP_LRPulseCountVTimeOut_flg_ovrdflg
      link override Signal_Override/_ovrdval: Value=KOUTP_LRPulseCountVTimeOut_flg_ovrdval
  VAPM_LRPulseCountV_flg_Inproc : FVT_lib/outp/OverrideAndLimit  SystemSampleTime=-1  VariantActivationTime=update diagram  Latency=0  AutoFrameSizeCalculation=off
      link override Signal_Limit/_maxval: Value=KOUTP_LRPulseCountV_flg_maxval
      link override Signal_Limit/_minval: Value=KOUTP_LRPulseCountV_flg_minval
      link override Signal_Override/_ovrdflg: Value=KOUTP_LRPulseCountV_flg_ovrdflg
      link override Signal_Override/_ovrdval: Value=KOUTP_LRPulseCountV_flg_ovrdval
  VAPM_LRPulseCount_enum_Inproc : FVT_lib/outp/OverrideAndLimit  SystemSampleTime=-1  VariantActivationTime=update diagram  Latency=0  AutoFrameSizeCalculation=off
      link override Signal_Limit/_maxval: Value=KOUTP_LRPulseCount_enum_maxval
      link override Signal_Limit/_minval: Value=KOUTP_LRPulseCount_enum_minval
      link override Signal_Override/_ovrdflg: Value=KOUTP_LRPulseCount_enum_ovrdflg
      link override Signal_Override/_ovrdval: Value=KOUTP_LRPulseCount_enum_ovrdval
  VAPM_LRRawWhlSpeedTimeOut_flg_Inproc : FVT_lib/outp/OverrideAndLimit  SystemSampleTime=-1  VariantActivationTime=update diagram  Latency=0  AutoFrameSizeCalculation=off
      link override Signal_Limit/_maxval: Value=KOUTP_LRRawWhlSpeedTimeOut_flg_maxval
      link override Signal_Limit/_minval: Value=KOUTP_LRRawWhlSpeedTimeOut_flg_minval
      link override Signal_Override/_ovrdflg: Value=KOUTP_LRRawWhlSpeedTimeOut_flg_ovrdflg
      link override Signal_Override/_ovrdval: Value=KOUTP_LRRawWhlSpeedTimeOut_flg_ovrdval
  VAPM_LRRawWhlSpeedVTimeOut_flg_Inproc : FVT_lib/outp/OverrideAndLimit  SystemSampleTime=-1  VariantActivationTime=update diagram  Latency=0  AutoFrameSizeCalculation=off
      link override Signal_Limit/_maxval: Value=KOUTP_LRRawWhlSpeedVTimeOut_flg_maxval
      link override Signal_Limit/_minval: Value=KOUTP_LRRawWhlSpeedVTimeOut_flg_minval
      link override Signal_Override/_ovrdflg: Value=KOUTP_LRRawWhlSpeedVTimeOut_flg_ovrdflg
      link override Signal_Override/_ovrdval: Value=KOUTP_LRRawWhlSpeedVTimeOut_flg_ovrdval
  VAPM_LRRawWhlSpeedV_flg_Inproc : FVT_lib/outp/OverrideAndLimit  SystemSampleTime=-1  VariantActivationTime=update diagram  Latency=0  AutoFrameSizeCalculation=off
      link override Signal_Limit/_maxval: Value=KOUTP_LRRawWhlSpeedV_flg_maxval
      link override Signal_Limit/_minval: Value=KOUTP_LRRawWhlSpeedV_flg_minval
      link override Signal_Override/_ovrdflg: Value=KOUTP_LRRawWhlSpeedV_flg_ovrdflg
      link override Signal_Override/_ovrdval: Value=KOUTP_LRRawWhlSpeedV_flg_ovrdval
  VAPM_LRRawWhlSpeed_kph_Inproc : FVT_lib/outp/OverrideAndLimit  SystemSampleTime=-1  VariantActivationTime=update diagram  Latency=0  AutoFrameSizeCalculation=off
      link override Signal_Limit/_maxval: Value=KOUTP_LRRawWhlSpeed_kph_maxval
      link override Signal_Limit/_minval: Value=KOUTP_LRRawWhlSpeed_kph_minval
      link override Signal_Override/_ovrdflg: Value=KOUTP_LRRawWhlSpeed_kph_ovrdflg
      link override Signal_Override/_ovrdval: Value=KOUTP_LRRawWhlSpeed_kph_ovrdval
  VAPM_LRWhlRotDirTimeOut_flg_Inproc : FVT_lib/outp/OverrideAndLimit  SystemSampleTime=-1  VariantActivationTime=update diagram  Latency=0  AutoFrameSizeCalculation=off
      link override Signal_Limit/_maxval: Value=KOUTP_LRWhlRotDirTimeOut_flg_maxval
      link override Signal_Limit/_minval: Value=KOUTP_LRWhlRotDirTimeOut_flg_minval
      link override Signal_Override/_ovrdflg: Value=KOUTP_LRWhlRotDirTimeOut_flg_ovrdflg
      link override Signal_Override/_ovrdval: Value=KOUTP_LRWhlRotDirTimeOut_flg_ovrdval
  VAPM_LRWhlRotDir_enum_Inproc : FVT_lib/outp/OverrideAndLimit  SystemSampleTime=-1  VariantActivationTime=update diagram  Latency=0  AutoFrameSizeCalculation=off
      link override Signal_Limit/_maxval: Value=KOUTP_LRWhlRotDir_enum_maxval
      link override Signal_Limit/_minval: Value=KOUTP_LRWhlRotDir_enum_minval
      link override Signal_Override/_ovrdflg: Value=KOUTP_LRWhlRotDir_enum_ovrdflg
      link override Signal_Override/_ovrdval: Value=KOUTP_LRWhlRotDir_enum_ovrdval
  VAPM_LatAccelTimeOut_flg_Inproc : FVT_lib/outp/OverrideAndLimit  SystemSampleTime=-1  VariantActivationTime=update diagram  Latency=0  AutoFrameSizeCalculation=off
      link override Signal_Limit/_maxval: Value=KOUTP_LatAccelTimeOut_flg_maxval
      link override Signal_Limit/_minval: Value=KOUTP_LatAccelTimeOut_flg_minval
      link override Signal_Override/_ovrdflg: Value=KOUTP_LatAccelTimeOut_flg_ovrdflg
      link override Signal_Override/_ovrdval: Value=KOUTP_LatAccelTimeOut_flg_ovrdval
  VAPM_LatAccelVTimeOut_flg_Inproc : FVT_lib/outp/OverrideAndLimit  SystemSampleTime=-1  VariantActivationTime=update diagram  Latency=0  AutoFrameSizeCalculation=off
      link override Signal_Limit/_maxval: Value=KOUTP_LatAccelVTimeOut_flg_maxval
      link override Signal_Limit/_minval: Value=KOUTP_LatAccelVTimeOut_flg_minval
      link override Signal_Override/_ovrdflg: Value=KOUTP_LatAccelVTimeOut_flg_ovrdflg
      link override Signal_Override/_ovrdval: Value=KOUTP_LatAccelVTimeOut_flg_ovrdval
  VAPM_LatAccelV_flg_Inproc : FVT_lib/outp/OverrideAndLimit  SystemSampleTime=-1  VariantActivationTime=update diagram  Latency=0  AutoFrameSizeCalculation=off
      link override Signal_Limit/_maxval: Value=KOUTP_LatAccelV_flg_maxval
      link override Signal_Limit/_minval: Value=KOUTP_LatAccelV_flg_minval
      link override Signal_Override/_ovrdflg: Value=KOUTP_LatAccelV_flg_ovrdflg
      link override Signal_Override/_ovrdval: Value=KOUTP_LatAccelV_flg_ovrdval
  VAPM_LatAccel_Gps_Inproc : FVT_lib/outp/OverrideAndLimit  SystemSampleTime=-1  VariantActivationTime=update diagram  Latency=0  AutoFrameSizeCalculation=off
      link override Signal_Limit/_maxval: Value=KOUTP_LatAccel_Gps_maxval
      link override Signal_Limit/_minval: Value=KOUTP_LatAccel_Gps_minval
      link override Signal_Override/_ovrdflg: Value=KOUTP_LatAccel_Gps_ovrdflg
      link override Signal_Override/_ovrdval: Value=KOUTP_LatAccel_Gps_ovrdval
  VAPM_LongAccelTimeOut_flg_Inproc : FVT_lib/outp/OverrideAndLimit  SystemSampleTime=-1  VariantActivationTime=update diagram  Latency=0  AutoFrameSizeCalculation=off
      link override Signal_Limit/_maxval: Value=KOUTP_LongAccelTimeOut_flg_maxval
      link override Signal_Limit/_minval: Value=KOUTP_LongAccelTimeOut_flg_minval
      link override Signal_Override/_ovrdflg: Value=KOUTP_LongAccelTimeOut_flg_ovrdflg
      link override Signal_Override/_ovrdval: Value=KOUTP_LongAccelTimeOut_flg_ovrdval
  VAPM_LongAccelVTimeOut_flg_Inproc : FVT_lib/outp/OverrideAndLimit  SystemSampleTime=-1  VariantActivationTime=update diagram  Latency=0  AutoFrameSizeCalculation=off
      link override Signal_Limit/_maxval: Value=KOUTP_LongAccelVTimeOut_flg_maxval
      link override Signal_Limit/_minval: Value=KOUTP_LongAccelVTimeOut_flg_minval
      link override Signal_Override/_ovrdflg: Value=KOUTP_LongAccelVTimeOut_flg_ovrdflg
      link override Signal_Override/_ovrdval: Value=KOUTP_LongAccelVTimeOut_flg_ovrdval
  VAPM_LongAccelV_flg_Inproc : FVT_lib/outp/OverrideAndLimit  SystemSampleTime=-1  VariantActivationTime=update diagram  Latency=0  AutoFrameSizeCalculation=off
      link override Signal_Limit/_maxval: Value=KOUTP_LongAccelV_flg_maxval
      link override Signal_Limit/_minval: Value=KOUTP_LongAccelV_flg_minval
      link override Signal_Override/_ovrdflg: Value=KOUTP_LongAccelV_flg_ovrdflg
      link override Signal_Override/_ovrdval: Value=KOUTP_LongAccelV_flg_ovrdval
  VAPM_LongAccel_Gps_Inproc : FVT_lib/outp/OverrideAndLimit  SystemSampleTime=-1  VariantActivationTime=update diagram  Latency=0  AutoFrameSizeCalculation=off
      link override Signal_Limit/_maxval: Value=KOUTP_LongAccel_Gps_maxval
      link override Signal_Limit/_minval: Value=KOUTP_LongAccel_Gps_minval
      link override Signal_Override/_ovrdflg: Value=KOUTP_LongAccel_Gps_ovrdflg
      link override Signal_Override/_ovrdval: Value=KOUTP_LongAccel_Gps_ovrdval
  VAPM_MCPressureTimeOut_flg_Inproc : FVT_lib/outp/OverrideAndLimit  SystemSampleTime=-1  VariantActivationTime=update diagram  Latency=0  AutoFrameSizeCalculation=off
      link override Signal_Limit/_maxval: Value=KOUTP_MCPressureTimeOut_flg_maxval
      link override Signal_Limit/_minval: Value=KOUTP_MCPressureTimeOut_flg_minval
      link override Signal_Override/_ovrdflg: Value=KOUTP_MCPressureTimeOut_flg_ovrdflg
      link override Signal_Override/_ovrdval: Value=KOUTP_MCPressureTimeOut_flg_ovrdval
  VAPM_MCPressureVTimeOut_flg_Inproc : FVT_lib/outp/OverrideAndLimit  SystemSampleTime=-1  VariantActivationTime=update diagram  Latency=0  AutoFrameSizeCalculation=off
      link override Signal_Limit/_maxval: Value=KOUTP_MCPressureVTimeOut_flg_maxval
      link override Signal_Limit/_minval: Value=KOUTP_MCPressureVTimeOut_flg_minval
      link override Signal_Override/_ovrdflg: Value=KOUTP_MCPressureVTimeOut_flg_ovrdflg
      link override Signal_Override/_ovrdval: Value=KOUTP_MCPressureVTimeOut_flg_ovrdval
  VAPM_MCPressureV_bar_Inproc : FVT_lib/outp/OverrideAndLimit  SystemSampleTime=-1  VariantActivationTime=update diagram  Latency=0  AutoFrameSizeCalculation=off
      link override Signal_Limit/_maxval: Value=KOUTP_MCPressureV_bar_maxval
      link override Signal_Limit/_minval: Value=KOUTP_MCPressureV_bar_minval
      link override Signal_Override/_ovrdflg: Value=KOUTP_MCPressureV_bar_ovrdflg
      link override Signal_Override/_ovrdval: Value=KOUTP_MCPressureV_bar_ovrdval
  VAPM_MCPressure_bar_Inproc : FVT_lib/outp/OverrideAndLimit  SystemSampleTime=-1  VariantActivationTime=update diagram  Latency=0  AutoFrameSizeCalculation=off
      link override Signal_Limit/_maxval: Value=KOUTP_MCPressure_bar_maxval
      link override Signal_Limit/_minval: Value=KOUTP_MCPressure_bar_minval
      link override Signal_Override/_ovrdflg: Value=KOUTP_MCPressure_bar_ovrdflg
      link override Signal_Override/_ovrdval: Value=KOUTP_MCPressure_bar_ovrdval
  VAPM_ModOperation_enum_Inproc : FVT_lib/outp/OverrideAndLimit  SystemSampleTime=-1  VariantActivationTime=update diagram  Latency=0  AutoFrameSizeCalculation=off
      link override Signal_Limit/_maxval: Value=KOUTP_ModOperation_enum_maxval
      link override Signal_Limit/_minval: Value=KOUTP_ModOperation_enum_minval
      link override Signal_Override/_ovrdflg: Value=KOUTP_ModOperation_enum_ovrdflg
      link override Signal_Override/_ovrdval: Value=KOUTP_ModOperation_enum_ovrdval
  VAPM_PASAFCL_enum_Inproc : FVT_lib/outp/OverrideAndLimit  SystemSampleTime=-1  VariantActivationTime=update diagram  Latency=0  AutoFrameSizeCalculation=off
      link override Signal_Limit/_maxval: Value=KOUTP_PASAFCL_enum_maxval
      link override Signal_Limit/_minval: Value=KOUTP_PASAFCL_enum_minval
      link override Signal_Override/_ovrdflg: Value=KOUTP_PASAFCL_enum_ovrdflg
      link override Signal_Override/_ovrdval: Value=KOUTP_PASAFCL_enum_ovrdval
  VAPM_PASAFCR_enum_Inproc : FVT_lib/outp/OverrideAndLimit  SystemSampleTime=-1  VariantActivationTime=update diagram  Latency=0  AutoFrameSizeCalculation=off
      link override Signal_Limit/_maxval: Value=KOUTP_PASAFCR_enum_maxval
      link override Signal_Limit/_minval: Value=KOUTP_PASAFCR_enum_minval
      link override Signal_Override/_ovrdflg: Value=KOUTP_PASAFCR_enum_ovrdflg
      link override Signal_Override/_ovrdval: Value=KOUTP_PASAFCR_enum_ovrdval
  VAPM_PASAFML_enum_Inproc : FVT_lib/outp/OverrideAndLimit  SystemSampleTime=-1  VariantActivationTime=update diagram  Latency=0  AutoFrameSizeCalculation=off
      link override Signal_Limit/_maxval: Value=KOUTP_PASAFML_enum_maxval
      link override Signal_Limit/_minval: Value=KOUTP_PASAFML_enum_minval
      link override Signal_Override/_ovrdflg: Value=KOUTP_PASAFML_enum_ovrdflg
      link override Signal_Override/_ovrdval: Value=KOUTP_PASAFML_enum_ovrdval
  VAPM_PASAFMR_enum_Inproc : FVT_lib/outp/OverrideAndLimit  SystemSampleTime=-1  VariantActivationTime=update diagram  Latency=0  AutoFrameSizeCalculation=off
      link override Signal_Limit/_maxval: Value=KOUTP_PASAFMR_enum_maxval
      link override Signal_Limit/_minval: Value=KOUTP_PASAFMR_enum_minval
      link override Signal_Override/_ovrdflg: Value=KOUTP_PASAFMR_enum_ovrdflg
      link override Signal_Override/_ovrdval: Value=KOUTP_PASAFMR_enum_ovrdval
  VAPM_PASARCL_enum_Inproc : FVT_lib/outp/OverrideAndLimit  SystemSampleTime=-1  VariantActivationTime=update diagram  Latency=0  AutoFrameSizeCalculation=off
      link override Signal_Limit/_maxval: Value=KOUTP_PASARCL_enum_maxval
      link override Signal_Limit/_minval: Value=KOUTP_PASARCL_enum_minval
      link override Signal_Override/_ovrdflg: Value=KOUTP_PASARCL_enum_ovrdflg
      link override Signal_Override/_ovrdval: Value=KOUTP_PASARCL_enum_ovrdval
  VAPM_PASARCR_enum_Inproc : FVT_lib/outp/OverrideAndLimit  SystemSampleTime=-1  VariantActivationTime=update diagram  Latency=0  AutoFrameSizeCalculation=off
      link override Signal_Limit/_maxval: Value=KOUTP_PASARCR_enum_maxval
      link override Signal_Limit/_minval: Value=KOUTP_PASARCR_enum_minval
      link override Signal_Override/_ovrdflg: Value=KOUTP_PASARCR_enum_ovrdflg
      link override Signal_Override/_ovrdval: Value=KOUTP_PASARCR_enum_ovrdval
  VAPM_PASARML_enum_Inproc : FVT_lib/outp/OverrideAndLimit  SystemSampleTime=-1  VariantActivationTime=update diagram  Latency=0  AutoFrameSizeCalculation=off
      link override Signal_Limit/_maxval: Value=KOUTP_PASARML_enum_maxval
      link override Signal_Limit/_minval: Value=KOUTP_PASARML_enum_minval
      link override Signal_Override/_ovrdflg: Value=KOUTP_PASARML_enum_ovrdflg
      link override Signal_Override/_ovrdval: Value=KOUTP_PASARML_enum_ovrdval
  VAPM_PASARMR_enum_Inproc : FVT_lib/outp/OverrideAndLimit  SystemSampleTime=-1  VariantActivationTime=update diagram  Latency=0  AutoFrameSizeCalculation=off
      link override Signal_Limit/_maxval: Value=KOUTP_PASARMR_enum_maxval
      link override Signal_Limit/_minval: Value=KOUTP_PASARMR_enum_minval
      link override Signal_Override/_ovrdflg: Value=KOUTP_PASARMR_enum_ovrdflg
      link override Signal_Override/_ovrdval: Value=KOUTP_PASARMR_enum_ovrdval
  VAPM_PASDFCL_cm_Inproc : FVT_lib/outp/OverrideAndLimit  SystemSampleTime=-1  VariantActivationTime=update diagram  Latency=0  AutoFrameSizeCalculation=off
      link override Signal_Limit/_maxval: Value=KOUTP_PASDFCL_cm_maxval
      link override Signal_Limit/_minval: Value=KOUTP_PASDFCL_cm_minval
      link override Signal_Override/_ovrdflg: Value=KOUTP_PASDFCL_cm_ovrdflg
      link override Signal_Override/_ovrdval: Value=KOUTP_PASDFCL_cm_ovrdval
  VAPM_PASDFCR_cm_Inproc : FVT_lib/outp/OverrideAndLimit  SystemSampleTime=-1  VariantActivationTime=update diagram  Latency=0  AutoFrameSizeCalculation=off
      link override Signal_Limit/_maxval: Value=KOUTP_PASDFCR_cm_maxval
      link override Signal_Limit/_minval: Value=KOUTP_PASDFCR_cm_minval
      link override Signal_Override/_ovrdflg: Value=KOUTP_PASDFCR_cm_ovrdflg
      link override Signal_Override/_ovrdval: Value=KOUTP_PASDFCR_cm_ovrdval
  VAPM_PASDFML_cm_Inproc : FVT_lib/outp/OverrideAndLimit  SystemSampleTime=-1  VariantActivationTime=update diagram  Latency=0  AutoFrameSizeCalculation=off
      link override Signal_Limit/_maxval: Value=KOUTP_PASDFML_cm_maxval
      link override Signal_Limit/_minval: Value=KOUTP_PASDFML_cm_minval
      link override Signal_Override/_ovrdflg: Value=KOUTP_PASDFML_cm_ovrdflg
      link override Signal_Override/_ovrdval: Value=KOUTP_PASDFML_cm_ovrdval
  VAPM_PASDFMR_cm_Inproc : FVT_lib/outp/OverrideAndLimit  SystemSampleTime=-1  VariantActivationTime=update diagram  Latency=0  AutoFrameSizeCalculation=off
      link override Signal_Limit/_maxval: Value=KOUTP_PASDFMR_cm_maxval
      link override Signal_Limit/_minval: Value=KOUTP_PASDFMR_cm_minval
      link override Signal_Override/_ovrdflg: Value=KOUTP_PASDFMR_cm_ovrdflg
      link override Signal_Override/_ovrdval: Value=KOUTP_PASDFMR_cm_ovrdval
  VAPM_PASDRCL_cm_Inproc : FVT_lib/outp/OverrideAndLimit  SystemSampleTime=-1  VariantActivationTime=update diagram  Latency=0  AutoFrameSizeCalculation=off
      link override Signal_Limit/_maxval: Value=KOUTP_PASDRCL_cm_maxval
      link override Signal_Limit/_minval: Value=KOUTP_PASDRCL_cm_minval
      link override Signal_Override/_ovrdflg: Value=KOUTP_PASDRCL_cm_ovrdflg
      link override Signal_Override/_ovrdval: Value=KOUTP_PASDRCL_cm_ovrdval
  VAPM_PASDRCR_cm_Inproc : FVT_lib/outp/OverrideAndLimit  SystemSampleTime=-1  VariantActivationTime=update diagram  Latency=0  AutoFrameSizeCalculation=off
      link override Signal_Limit/_maxval: Value=KOUTP_PASDRCR_cm_maxval
      link override Signal_Limit/_minval: Value=KOUTP_PASDRCR_cm_minval
      link override Signal_Override/_ovrdflg: Value=KOUTP_PASDRCR_cm_ovrdflg
      link override Signal_Override/_ovrdval: Value=KOUTP_PASDRCR_cm_ovrdval
  VAPM_PASDRML_cm_Inproc : FVT_lib/outp/OverrideAndLimit  SystemSampleTime=-1  VariantActivationTime=update diagram  Latency=0  AutoFrameSizeCalculation=off
      link override Signal_Limit/_maxval: Value=KOUTP_PASDRML_cm_maxval
      link override Signal_Limit/_minval: Value=KOUTP_PASDRML_cm_minval
      link override Signal_Override/_ovrdflg: Value=KOUTP_PASDRML_cm_ovrdflg
      link override Signal_Override/_ovrdval: Value=KOUTP_PASDRML_cm_ovrdval
  VAPM_PASDRMR_cm_Inproc : FVT_lib/outp/OverrideAndLimit  SystemSampleTime=-1  VariantActivationTime=update diagram  Latency=0  AutoFrameSizeCalculation=off
      link override Signal_Limit/_maxval: Value=KOUTP_PASDRMR_cm_maxval
      link override Signal_Limit/_minval: Value=KOUTP_PASDRMR_cm_minval
      link override Signal_Override/_ovrdflg: Value=KOUTP_PASDRMR_cm_ovrdflg
      link override Signal_Override/_ovrdval: Value=KOUTP_PASDRMR_cm_ovrdval
  VAPM_RFPulseCountTimeOut_flg_Inproc : FVT_lib/outp/OverrideAndLimit  SystemSampleTime=-1  VariantActivationTime=update diagram  Latency=0  AutoFrameSizeCalculation=off
      link override Signal_Limit/_maxval: Value=KOUTP_RFPulseCountTimeOut_flg_maxval
      link override Signal_Limit/_minval: Value=KOUTP_RFPulseCountTimeOut_flg_minval
      link override Signal_Override/_ovrdflg: Value=KOUTP_RFPulseCountTimeOut_flg_ovrdflg
      link override Signal_Override/_ovrdval: Value=KOUTP_RFPulseCountTimeOut_flg_ovrdval
  VAPM_RFPulseCountVTimeOut_flg_Inproc : FVT_lib/outp/OverrideAndLimit  SystemSampleTime=-1  VariantActivationTime=update diagram  Latency=0  AutoFrameSizeCalculation=off
      link override Signal_Limit/_maxval: Value=KOUTP_RFPulseCountVTimeOut_flg_maxval
      link override Signal_Limit/_minval: Value=KOUTP_RFPulseCountVTimeOut_flg_minval
      link override Signal_Override/_ovrdflg: Value=KOUTP_RFPulseCountVTimeOut_flg_ovrdflg
      link override Signal_Override/_ovrdval: Value=KOUTP_RFPulseCountVTimeOut_flg_ovrdval
  VAPM_RFPulseCountV_flg_Inproc : FVT_lib/outp/OverrideAndLimit  SystemSampleTime=-1  VariantActivationTime=update diagram  Latency=0  AutoFrameSizeCalculation=off
      link override Signal_Limit/_maxval: Value=KOUTP_RFPulseCountV_flg_maxval
      link override Signal_Limit/_minval: Value=KOUTP_RFPulseCountV_flg_minval
      link override Signal_Override/_ovrdflg: Value=KOUTP_RFPulseCountV_flg_ovrdflg
      link override Signal_Override/_ovrdval: Value=KOUTP_RFPulseCountV_flg_ovrdval
  VAPM_RFPulseCount_enum_Inproc : FVT_lib/outp/OverrideAndLimit  SystemSampleTime=-1  VariantActivationTime=update diagram  Latency=0  AutoFrameSizeCalculation=off
      link override Signal_Limit/_maxval: Value=KOUTP_RFPulseCount_enum_maxval
      link override Signal_Limit/_minval: Value=KOUTP_RFPulseCount_enum_minval
      link override Signal_Override/_ovrdflg: Value=KOUTP_RFPulseCount_enum_ovrdflg
      link override Signal_Override/_ovrdval: Value=KOUTP_RFPulseCount_enum_ovrdval
  VAPM_RFRawWhlSpeedTimeOut_flg_Inproc : FVT_lib/outp/OverrideAndLimit  SystemSampleTime=-1  VariantActivationTime=update diagram  Latency=0  AutoFrameSizeCalculation=off
      link override Signal_Limit/_maxval: Value=KOUTP_RFRawWhlSpeedTimeOut_flg_maxval
      link override Signal_Limit/_minval: Value=KOUTP_RFRawWhlSpeedTimeOut_flg_minval
      link override Signal_Override/_ovrdflg: Value=KOUTP_RFRawWhlSpeedTimeOut_flg_ovrdflg
      link override Signal_Override/_ovrdval: Value=KOUTP_RFRawWhlSpeedTimeOut_flg_ovrdval
  VAPM_RFRawWhlSpeedVTimeOut_flg_Inproc : FVT_lib/outp/OverrideAndLimit  SystemSampleTime=-1  VariantActivationTime=update diagram  Latency=0  AutoFrameSizeCalculation=off
      link override Signal_Limit/_maxval: Value=KOUTP_RFRawWhlSpeedVTimeOut_flg_maxval
      link override Signal_Limit/_minval: Value=KOUTP_RFRawWhlSpeedVTimeOut_flg_minval
      link override Signal_Override/_ovrdflg: Value=KOUTP_RFRawWhlSpeedVTimeOut_flg_ovrdflg
      link override Signal_Override/_ovrdval: Value=KOUTP_RFRawWhlSpeedVTimeOut_flg_ovrdval
  VAPM_RFRawWhlSpeedV_flg_Inproc : FVT_lib/outp/OverrideAndLimit  SystemSampleTime=-1  VariantActivationTime=update diagram  Latency=0  AutoFrameSizeCalculation=off
      link override Signal_Limit/_maxval: Value=KOUTP_RFRawWhlSpeedV_flg_maxval
      link override Signal_Limit/_minval: Value=KOUTP_RFRawWhlSpeedV_flg_minval
      link override Signal_Override/_ovrdflg: Value=KOUTP_RFRawWhlSpeedV_flg_ovrdflg
      link override Signal_Override/_ovrdval: Value=KOUTP_RFRawWhlSpeedV_flg_ovrdval
  VAPM_RFRawWhlSpeed_kph_Inproc : FVT_lib/outp/OverrideAndLimit  SystemSampleTime=-1  VariantActivationTime=update diagram  Latency=0  AutoFrameSizeCalculation=off
      link override Signal_Limit/_maxval: Value=KOUTP_RFRawWhlSpeed_kph_maxval
      link override Signal_Limit/_minval: Value=KOUTP_RFRawWhlSpeed_kph_minval
      link override Signal_Override/_ovrdflg: Value=KOUTP_RFRawWhlSpeed_kph_ovrdflg
      link override Signal_Override/_ovrdval: Value=KOUTP_RFRawWhlSpeed_kph_ovrdval
  VAPM_RFWhlRotDirTimeOut_flg_Inproc : FVT_lib/outp/OverrideAndLimit  SystemSampleTime=-1  VariantActivationTime=update diagram  Latency=0  AutoFrameSizeCalculation=off
      link override Signal_Limit/_maxval: Value=KOUTP_RFWhlRotDirTimeOut_flg_maxval
      link override Signal_Limit/_minval: Value=KOUTP_RFWhlRotDirTimeOut_flg_minval
      link override Signal_Override/_ovrdflg: Value=KOUTP_RFWhlRotDirTimeOut_flg_ovrdflg
      link override Signal_Override/_ovrdval: Value=KOUTP_RFWhlRotDirTimeOut_flg_ovrdval
  VAPM_RFWhlRotDir_enum_Inproc : FVT_lib/outp/OverrideAndLimit  SystemSampleTime=-1  VariantActivationTime=update diagram  Latency=0  AutoFrameSizeCalculation=off
      link override Signal_Limit/_maxval: Value=KOUTP_RFWhlRotDir_enum_maxval
      link override Signal_Limit/_minval: Value=KOUTP_RFWhlRotDir_enum_minval
      link override Signal_Override/_ovrdflg: Value=KOUTP_RFWhlRotDir_enum_ovrdflg
      link override Signal_Override/_ovrdval: Value=KOUTP_RFWhlRotDir_enum_ovrdval
  VAPM_RRPulseCountTimeOut_flg_Inproc : FVT_lib/outp/OverrideAndLimit  SystemSampleTime=-1  VariantActivationTime=update diagram  Latency=0  AutoFrameSizeCalculation=off
      link override Signal_Limit/_maxval: Value=KOUTP_RRPulseCountTimeOut_flg_maxval
      link override Signal_Limit/_minval: Value=KOUTP_RRPulseCountTimeOut_flg_minval
      link override Signal_Override/_ovrdflg: Value=KOUTP_RRPulseCountTimeOut_flg_ovrdflg
      link override Signal_Override/_ovrdval: Value=KOUTP_RRPulseCountTimeOut_flg_ovrdval
  VAPM_RRPulseCountVTimeOut_flg_Inproc : FVT_lib/outp/OverrideAndLimit  SystemSampleTime=-1  VariantActivationTime=update diagram  Latency=0  AutoFrameSizeCalculation=off
      link override Signal_Limit/_maxval: Value=KOUTP_RRPulseCountVTimeOut_flg_maxval
      link override Signal_Limit/_minval: Value=KOUTP_RRPulseCountVTimeOut_flg_minval
      link override Signal_Override/_ovrdflg: Value=KOUTP_RRPulseCountVTimeOut_flg_ovrdflg
      link override Signal_Override/_ovrdval: Value=KOUTP_RRPulseCountVTimeOut_flg_ovrdval
  VAPM_RRPulseCountV_flg_Inproc : FVT_lib/outp/OverrideAndLimit  SystemSampleTime=-1  VariantActivationTime=update diagram  Latency=0  AutoFrameSizeCalculation=off
      link override Signal_Limit/_maxval: Value=KOUTP_RRPulseCountV_flg_maxval
      link override Signal_Limit/_minval: Value=KOUTP_RRPulseCountV_flg_minval
      link override Signal_Override/_ovrdflg: Value=KOUTP_RRPulseCountV_flg_ovrdflg
      link override Signal_Override/_ovrdval: Value=KOUTP_RRPulseCountV_flg_ovrdval
  VAPM_RRPulseCount_enum_Inproc : FVT_lib/outp/OverrideAndLimit  SystemSampleTime=-1  VariantActivationTime=update diagram  Latency=0  AutoFrameSizeCalculation=off
      link override Signal_Limit/_maxval: Value=KOUTP_RRPulseCount_enum_maxval
      link override Signal_Limit/_minval: Value=KOUTP_RRPulseCount_enum_minval
      link override Signal_Override/_ovrdflg: Value=KOUTP_RRPulseCount_enum_ovrdflg
      link override Signal_Override/_ovrdval: Value=KOUTP_RRPulseCount_enum_ovrdval
  VAPM_RRRawWhlSpeedTimeOut_flg_Inproc : FVT_lib/outp/OverrideAndLimit  SystemSampleTime=-1  VariantActivationTime=update diagram  Latency=0  AutoFrameSizeCalculation=off
      link override Signal_Limit/_maxval: Value=KOUTP_RRRawWhlSpeedTimeOut_flg_maxval
      link override Signal_Limit/_minval: Value=KOUTP_RRRawWhlSpeedTimeOut_flg_minval
      link override Signal_Override/_ovrdflg: Value=KOUTP_RRRawWhlSpeedTimeOut_flg_ovrdflg
      link override Signal_Override/_ovrdval: Value=KOUTP_RRRawWhlSpeedTimeOut_flg_ovrdval
  VAPM_RRRawWhlSpeedVTimeOut_flg_Inproc : FVT_lib/outp/OverrideAndLimit  SystemSampleTime=-1  VariantActivationTime=update diagram  Latency=0  AutoFrameSizeCalculation=off
      link override Signal_Limit/_maxval: Value=KOUTP_RRRawWhlSpeedVTimeOut_flg_maxval
      link override Signal_Limit/_minval: Value=KOUTP_RRRawWhlSpeedVTimeOut_flg_minval
      link override Signal_Override/_ovrdflg: Value=KOUTP_RRRawWhlSpeedVTimeOut_flg_ovrdflg
      link override Signal_Override/_ovrdval: Value=KOUTP_RRRawWhlSpeedVTimeOut_flg_ovrdval
  VAPM_RRRawWhlSpeedV_flg_Inproc : FVT_lib/outp/OverrideAndLimit  SystemSampleTime=-1  VariantActivationTime=update diagram  Latency=0  AutoFrameSizeCalculation=off
      link override Signal_Limit/_maxval: Value=KOUTP_RRRawWhlSpeedV_flg_maxval
      link override Signal_Limit/_minval: Value=KOUTP_RRRawWhlSpeedV_flg_minval
      link override Signal_Override/_ovrdflg: Value=KOUTP_RRRawWhlSpeedV_flg_ovrdflg
      link override Signal_Override/_ovrdval: Value=KOUTP_RRRawWhlSpeedV_flg_ovrdval
  VAPM_RRRawWhlSpeed_kph_Inproc : FVT_lib/outp/OverrideAndLimit  SystemSampleTime=-1  VariantActivationTime=update diagram  Latency=0  AutoFrameSizeCalculation=off
      link override Signal_Limit/_maxval: Value=KOUTP_RRRawWhlSpeed_kph_maxval
      link override Signal_Limit/_minval: Value=KOUTP_RRRawWhlSpeed_kph_minval
      link override Signal_Override/_ovrdflg: Value=KOUTP_RRRawWhlSpeed_kph_ovrdflg
      link override Signal_Override/_ovrdval: Value=KOUTP_RRRawWhlSpeed_kph_ovrdval
  VAPM_RRWhlRotDirTimeOut_flg_Inproc : FVT_lib/outp/OverrideAndLimit  SystemSampleTime=-1  VariantActivationTime=update diagram  Latency=0  AutoFrameSizeCalculation=off
      link override Signal_Limit/_maxval: Value=KOUTP_RRWhlRotDirTimeOut_flg_maxval
      link override Signal_Limit/_minval: Value=KOUTP_RRWhlRotDirTimeOut_flg_minval
      link override Signal_Override/_ovrdflg: Value=KOUTP_RRWhlRotDirTimeOut_flg_ovrdflg
      link override Signal_Override/_ovrdval: Value=KOUTP_RRWhlRotDirTimeOut_flg_ovrdval
  VAPM_RRWhlRotDir_enum_Inproc : FVT_lib/outp/OverrideAndLimit  SystemSampleTime=-1  VariantActivationTime=update diagram  Latency=0  AutoFrameSizeCalculation=off
      link override Signal_Limit/_maxval: Value=KOUTP_RRWhlRotDir_enum_maxval
      link override Signal_Limit/_minval: Value=KOUTP_RRWhlRotDir_enum_minval
      link override Signal_Override/_ovrdflg: Value=KOUTP_RRWhlRotDir_enum_ovrdflg
      link override Signal_Override/_ovrdval: Value=KOUTP_RRWhlRotDir_enum_ovrdval
  VAPM_SASAngleTimeOut_flg_Inproc : FVT_lib/outp/OverrideAndLimit  SystemSampleTime=-1  VariantActivationTime=update diagram  Latency=0  AutoFrameSizeCalculation=off
      link override Signal_Limit/_maxval: Value=KOUTP_SASAngleTimeOut_flg_maxval
      link override Signal_Limit/_minval: Value=KOUTP_SASAngleTimeOut_flg_minval
      link override Signal_Override/_ovrdflg: Value=KOUTP_SASAngleTimeOut_flg_ovrdflg
      link override Signal_Override/_ovrdval: Value=KOUTP_SASAngleTimeOut_flg_ovrdval
  VAPM_SASAngle_Deg_Inproc : FVT_lib/outp/OverrideAndLimit  SystemSampleTime=-1  VariantActivationTime=update diagram  Latency=0  AutoFrameSizeCalculation=off
      link override Signal_Limit/_maxval: Value=KOUTP_SASAngle_Deg_maxval
      link override Signal_Limit/_minval: Value=KOUTP_SASAngle_Deg_minval
      link override Signal_Override/_ovrdflg: Value=KOUTP_SASAngle_Deg_ovrdflg
      link override Signal_Override/_ovrdval: Value=KOUTP_SASAngle_Deg_ovrdval
  VAPM_SASCALTimeOut_flg_Inproc : FVT_lib/outp/OverrideAndLimit  SystemSampleTime=-1  VariantActivationTime=update diagram  Latency=0  AutoFrameSizeCalculation=off
      link override Signal_Limit/_maxval: Value=KOUTP_SASCALTimeOut_flg_maxval
      link override Signal_Limit/_minval: Value=KOUTP_SASCALTimeOut_flg_minval
      link override Signal_Override/_ovrdflg: Value=KOUTP_SASCALTimeOut_flg_ovrdflg
      link override Signal_Override/_ovrdval: Value=KOUTP_SASCALTimeOut_flg_ovrdval
  VAPM_SASCAL_flg_Inproc : FVT_lib/outp/OverrideAndLimit  SystemSampleTime=-1  VariantActivationTime=update diagram  Latency=0  AutoFrameSizeCalculation=off
      link override Signal_Limit/_maxval: Value=KOUTP_SASCAL_flg_maxval
      link override Signal_Limit/_minval: Value=KOUTP_SASCAL_flg_minval
      link override Signal_Override/_ovrdflg: Value=KOUTP_SASCAL_flg_ovrdflg
      link override Signal_Override/_ovrdval: Value=KOUTP_SASCAL_flg_ovrdval
  VAPM_SASSpeedTimeOut_flg_Inproc : FVT_lib/outp/OverrideAndLimit  SystemSampleTime=-1  VariantActivationTime=update diagram  Latency=0  AutoFrameSizeCalculation=off
      link override Signal_Limit/_maxval: Value=KOUTP_SASSpeedTimeOut_flg_maxval
      link override Signal_Limit/_minval: Value=KOUTP_SASSpeedTimeOut_flg_minval
      link override Signal_Override/_ovrdflg: Value=KOUTP_SASSpeedTimeOut_flg_ovrdflg
      link override Signal_Override/_ovrdval: Value=KOUTP_SASSpeedTimeOut_flg_ovrdval
  VAPM_SASSpeedValidTimeOut_flg_Inproc : FVT_lib/outp/OverrideAndLimit  SystemSampleTime=-1  VariantActivationTime=update diagram  Latency=0  AutoFrameSizeCalculation=off
      link override Signal_Limit/_maxval: Value=KOUTP_SASSpeedValidTimeOut_flg_maxval
      link override Signal_Limit/_minval: Value=KOUTP_SASSpeedValidTimeOut_flg_minval
      link override Signal_Override/_ovrdflg: Value=KOUTP_SASSpeedValidTimeOut_flg_ovrdflg
      link override Signal_Override/_ovrdval: Value=KOUTP_SASSpeedValidTimeOut_flg_ovrdval
  VAPM_SASSpeedValid_flg_Inproc : FVT_lib/outp/OverrideAndLimit  SystemSampleTime=-1  VariantActivationTime=update diagram  Latency=0  AutoFrameSizeCalculation=off
      link override Signal_Limit/_maxval: Value=KOUTP_SASSpeedValid_flg_maxval
      link override Signal_Limit/_minval: Value=KOUTP_SASSpeedValid_flg_minval
      link override Signal_Override/_ovrdflg: Value=KOUTP_SASSpeedValid_flg_ovrdflg
      link override Signal_Override/_ovrdval: Value=KOUTP_SASSpeedValid_flg_ovrdval
  VAPM_SASSpeed_degps_Inproc : FVT_lib/outp/OverrideAndLimit  SystemSampleTime=-1  VariantActivationTime=update diagram  Latency=0  AutoFrameSizeCalculation=off
      link override Signal_Limit/_maxval: Value=KOUTP_SASSpeed_degps_maxval
      link override Signal_Limit/_minval: Value=KOUTP_SASSpeed_degps_minval
      link override Signal_Override/_ovrdflg: Value=KOUTP_SASSpeed_degps_ovrdflg
      link override Signal_Override/_ovrdval: Value=KOUTP_SASSpeed_degps_ovrdval
  VAPM_SASVTimeOut_flg_Inproc : FVT_lib/outp/OverrideAndLimit  SystemSampleTime=-1  VariantActivationTime=update diagram  Latency=0  AutoFrameSizeCalculation=off
      link override Signal_Limit/_maxval: Value=KOUTP_SASVTimeOut_flg_maxval
      link override Signal_Limit/_minval: Value=KOUTP_SASVTimeOut_flg_minval
      link override Signal_Override/_ovrdflg: Value=KOUTP_SASVTimeOut_flg_ovrdflg
      link override Signal_Override/_ovrdval: Value=KOUTP_SASVTimeOut_flg_ovrdval
  VAPM_SASV_flg_Inproc : FVT_lib/outp/OverrideAndLimit  SystemSampleTime=-1  VariantActivationTime=update diagram  Latency=0  AutoFrameSizeCalculation=off
      link override Signal_Limit/_maxval: Value=KOUTP_SASV_flg_maxval
      link override Signal_Limit/_minval: Value=KOUTP_SASV_flg_minval
      link override Signal_Override/_ovrdflg: Value=KOUTP_SASV_flg_ovrdflg
      link override Signal_Override/_ovrdval: Value=KOUTP_SASV_flg_ovrdval
  VAPM_SNSRLayout_enum_Inproc : FVT_lib/outp/OverrideAndLimit  SystemSampleTime=-1  VariantActivationTime=update diagram  Latency=0  AutoFrameSizeCalculation=off
      link override Signal_Limit/_maxval: Value=KOUTP_SNSRLayout_enum_maxval
      link override Signal_Limit/_minval: Value=KOUTP_SNSRLayout_enum_minval
      link override Signal_Override/_ovrdflg: Value=KOUTP_SNSRLayout_enum_ovrdflg
      link override Signal_Override/_ovrdval: Value=KOUTP_SNSRLayout_enum_ovrdval
  VAPM_ShifterHandleCmdTimeOut_flg_Inproc : FVT_lib/outp/OverrideAndLimit  SystemSampleTime=-1  VariantActivationTime=update diagram  Latency=0  AutoFrameSizeCalculation=off
      link override Signal_Limit/_maxval: Value=KOUTP_ShifterHandleCmdTimeOut_flg_maxval
      link override Signal_Limit/_minval: Value=KOUTP_ShifterHandleCmdTimeOut_flg_minval
      link override Signal_Override/_ovrdflg: Value=KOUTP_ShifterHandleCmdTimeOut_flg_ovrdflg
      link override Signal_Override/_ovrdval: Value=KOUTP_ShifterHandleCmdTimeOut_flg_ovrdval
  VAPM_ShifterHandleCmd_enum_Inproc : FVT_lib/outp/OverrideAndLimit  SystemSampleTime=-1  VariantActivationTime=update diagram  Latency=0  AutoFrameSizeCalculation=off
      link override Signal_Limit/_maxval: Value=KOUTP_ShifterHandleCmd_enum_maxval
      link override Signal_Limit/_minval: Value=KOUTP_ShifterHandleCmd_enum_minval
      link override Signal_Override/_ovrdflg: Value=KOUTP_ShifterHandleCmd_enum_ovrdflg
      link override Signal_Override/_ovrdval: Value=KOUTP_ShifterHandleCmd_enum_ovrdval
  VAPM_StaFSya_flg_Inproc : FVT_lib/outp/OverrideAndLimit  SystemSampleTime=-1  VariantActivationTime=update diagram  Latency=0  AutoFrameSizeCalculation=off
      link override Signal_Limit/_maxval: Value=KOUTP_StaFSya_flg_maxval
      link override Signal_Limit/_minval: Value=KOUTP_StaFSya_flg_minval
      link override Signal_Override/_ovrdflg: Value=KOUTP_StaFSya_flg_ovrdflg
      link override Signal_Override/_ovrdval: Value=KOUTP_StaFSya_flg_ovrdval
  VAPM_TCSActiveTimeOut_flg_Inproc : FVT_lib/outp/OverrideAndLimit  SystemSampleTime=-1  VariantActivationTime=update diagram  Latency=0  AutoFrameSizeCalculation=off
      link override Signal_Limit/_maxval: Value=KOUTP_TCSActiveTimeOut_flg_maxval
      link override Signal_Limit/_minval: Value=KOUTP_TCSActiveTimeOut_flg_minval
      link override Signal_Override/_ovrdflg: Value=KOUTP_TCSActiveTimeOut_flg_ovrdflg
      link override Signal_Override/_ovrdval: Value=KOUTP_TCSActiveTimeOut_flg_ovrdval
  VAPM_TCSActiveToAPM_flg_Inproc : FVT_lib/outp/OverrideAndLimit  SystemSampleTime=-1  VariantActivationTime=update diagram  Latency=0  AutoFrameSizeCalculation=off
      link override Signal_Limit/_maxval: Value=KOUTP_TCSActiveToAPM_flg_maxval
      link override Signal_Limit/_minval: Value=KOUTP_TCSActiveToAPM_flg_minval
      link override Signal_Override/_ovrdflg: Value=KOUTP_TCSActiveToAPM_flg_ovrdflg
      link override Signal_Override/_ovrdval: Value=KOUTP_TCSActiveToAPM_flg_ovrdval
  VAPM_USSStaFCL_flg_Inproc : FVT_lib/outp/OverrideAndLimit  SystemSampleTime=-1  VariantActivationTime=update diagram  Latency=0  AutoFrameSizeCalculation=off
      link override Signal_Limit/_maxval: Value=KOUTP_USSStaFCL_flg_maxval
      link override Signal_Limit/_minval: Value=KOUTP_USSStaFCL_flg_minval
      link override Signal_Override/_ovrdflg: Value=KOUTP_USSStaFCL_flg_ovrdflg
      link override Signal_Override/_ovrdval: Value=KOUTP_USSStaFCL_flg_ovrdval
  VAPM_USSStaFCR_flg_Inproc : FVT_lib/outp/OverrideAndLimit  SystemSampleTime=-1  VariantActivationTime=update diagram  Latency=0  AutoFrameSizeCalculation=off
      link override Signal_Limit/_maxval: Value=KOUTP_USSStaFCR_flg_maxval
      link override Signal_Limit/_minval: Value=KOUTP_USSStaFCR_flg_minval
      link override Signal_Override/_ovrdflg: Value=KOUTP_USSStaFCR_flg_ovrdflg
      link override Signal_Override/_ovrdval: Value=KOUTP_USSStaFCR_flg_ovrdval
  VAPM_USSStaFLL_flg_Inproc : FVT_lib/outp/OverrideAndLimit  SystemSampleTime=-1  VariantActivationTime=update diagram  Latency=0  AutoFrameSizeCalculation=off
      link override Signal_Limit/_maxval: Value=KOUTP_USSStaFLL_flg_maxval
      link override Signal_Limit/_minval: Value=KOUTP_USSStaFLL_flg_minval
      link override Signal_Override/_ovrdflg: Value=KOUTP_USSStaFLL_flg_ovrdflg
      link override Signal_Override/_ovrdval: Value=KOUTP_USSStaFLL_flg_ovrdval
  VAPM_USSStaFLR_flg_Inproc : FVT_lib/outp/OverrideAndLimit  SystemSampleTime=-1  VariantActivationTime=update diagram  Latency=0  AutoFrameSizeCalculation=off
      link override Signal_Limit/_maxval: Value=KOUTP_USSStaFLR_flg_maxval
      link override Signal_Limit/_minval: Value=KOUTP_USSStaFLR_flg_minval
      link override Signal_Override/_ovrdflg: Value=KOUTP_USSStaFLR_flg_ovrdflg
      link override Signal_Override/_ovrdval: Value=KOUTP_USSStaFLR_flg_ovrdval
  VAPM_USSStaFML_flg_Inproc : FVT_lib/outp/OverrideAndLimit  SystemSampleTime=-1  VariantActivationTime=update diagram  Latency=0  AutoFrameSizeCalculation=off
      link override Signal_Limit/_maxval: Value=KOUTP_USSStaFML_flg_maxval
      link override Signal_Limit/_minval: Value=KOUTP_USSStaFML_flg_minval
      link override Signal_Override/_ovrdflg: Value=KOUTP_USSStaFML_flg_ovrdflg
      link override Signal_Override/_ovrdval: Value=KOUTP_USSStaFML_flg_ovrdval
  VAPM_USSStaFMR_flg_Inproc : FVT_lib/outp/OverrideAndLimit  SystemSampleTime=-1  VariantActivationTime=update diagram  Latency=0  AutoFrameSizeCalculation=off
      link override Signal_Limit/_maxval: Value=KOUTP_USSStaFMR_flg_maxval
      link override Signal_Limit/_minval: Value=KOUTP_USSStaFMR_flg_minval
      link override Signal_Override/_ovrdflg: Value=KOUTP_USSStaFMR_flg_ovrdflg
      link override Signal_Override/_ovrdval: Value=KOUTP_USSStaFMR_flg_ovrdval
  VAPM_USSStaRCL_flg_Inproc : FVT_lib/outp/OverrideAndLimit  SystemSampleTime=-1  VariantActivationTime=update diagram  Latency=0  AutoFrameSizeCalculation=off
      link override Signal_Limit/_maxval: Value=KOUTP_USSStaRCL_flg_maxval
      link override Signal_Limit/_minval: Value=KOUTP_USSStaRCL_flg_minval
      link override Signal_Override/_ovrdflg: Value=KOUTP_USSStaRCL_flg_ovrdflg
      link override Signal_Override/_ovrdval: Value=KOUTP_USSStaRCL_flg_ovrdval
  VAPM_USSStaRCR_flg_Inproc : FVT_lib/outp/OverrideAndLimit  SystemSampleTime=-1  VariantActivationTime=update diagram  Latency=0  AutoFrameSizeCalculation=off
      link override Signal_Limit/_maxval: Value=KOUTP_USSStaRCR_flg_maxval
      link override Signal_Limit/_minval: Value=KOUTP_USSStaRCR_flg_minval
      link override Signal_Override/_ovrdflg: Value=KOUTP_USSStaRCR_flg_ovrdflg
      link override Signal_Override/_ovrdval: Value=KOUTP_USSStaRCR_flg_ovrdval
  VAPM_USSStaRLL_flg_Inproc : FVT_lib/outp/OverrideAndLimit  SystemSampleTime=-1  VariantActivationTime=update diagram  Latency=0  AutoFrameSizeCalculation=off
      link override Signal_Limit/_maxval: Value=KOUTP_USSStaRLL_flg_maxval
      link override Signal_Limit/_minval: Value=KOUTP_USSStaRLL_flg_minval
      link override Signal_Override/_ovrdflg: Value=KOUTP_USSStaRLL_flg_ovrdflg
      link override Signal_Override/_ovrdval: Value=KOUTP_USSStaRLL_flg_ovrdval
  VAPM_USSStaRLR_flg_Inproc : FVT_lib/outp/OverrideAndLimit  SystemSampleTime=-1  VariantActivationTime=update diagram  Latency=0  AutoFrameSizeCalculation=off
      link override Signal_Limit/_maxval: Value=KOUTP_USSStaRLR_flg_maxval
      link override Signal_Limit/_minval: Value=KOUTP_USSStaRLR_flg_minval
      link override Signal_Override/_ovrdflg: Value=KOUTP_USSStaRLR_flg_ovrdflg
      link override Signal_Override/_ovrdval: Value=KOUTP_USSStaRLR_flg_ovrdval
  VAPM_USSStaRML_flg_Inproc : FVT_lib/outp/OverrideAndLimit  SystemSampleTime=-1  VariantActivationTime=update diagram  Latency=0  AutoFrameSizeCalculation=off
      link override Signal_Limit/_maxval: Value=KOUTP_USSStaRML_flg_maxval
      link override Signal_Limit/_minval: Value=KOUTP_USSStaRML_flg_minval
      link override Signal_Override/_ovrdflg: Value=KOUTP_USSStaRML_flg_ovrdflg
      link override Signal_Override/_ovrdval: Value=KOUTP_USSStaRML_flg_ovrdval
  VAPM_USSStaRMR_flg_Inproc : FVT_lib/outp/OverrideAndLimit  SystemSampleTime=-1  VariantActivationTime=update diagram  Latency=0  AutoFrameSizeCalculation=off
      link override Signal_Limit/_maxval: Value=KOUTP_USSStaRMR_flg_maxval
      link override Signal_Limit/_minval: Value=KOUTP_USSStaRMR_flg_minval
      link override Signal_Override/_ovrdflg: Value=KOUTP_USSStaRMR_flg_ovrdflg
      link override Signal_Override/_ovrdval: Value=KOUTP_USSStaRMR_flg_ovrdval
  VAPM_VehSpeedTimeOut_flg_Inproc : FVT_lib/outp/OverrideAndLimit  SystemSampleTime=-1  VariantActivationTime=update diagram  Latency=0  AutoFrameSizeCalculation=off
      link override Signal_Limit/_maxval: Value=KOUTP_VehSpeedTimeOut_flg_maxval
      link override Signal_Limit/_minval: Value=KOUTP_VehSpeedTimeOut_flg_minval
      link override Signal_Override/_ovrdflg: Value=KOUTP_VehSpeedTimeOut_flg_ovrdflg
      link override Signal_Override/_ovrdval: Value=KOUTP_VehSpeedTimeOut_flg_ovrdval
  VAPM_VehSpeedToAPM_kph_Inproc : FVT_lib/outp/OverrideAndLimit  SystemSampleTime=-1  VariantActivationTime=update diagram  Latency=0  AutoFrameSizeCalculation=off
      link override Signal_Limit/_maxval: Value=KOUTP_VehSpeedToAPM_kph_maxval
      link override Signal_Limit/_minval: Value=KOUTP_VehSpeedToAPM_kph_minval
      link override Signal_Override/_ovrdflg: Value=KOUTP_VehSpeedToAPM_kph_ovrdflg
      link override Signal_Override/_ovrdval: Value=KOUTP_VehSpeedToAPM_kph_ovrdval
  VAPM_YawRateTimeOut_flg_Inproc : FVT_lib/outp/OverrideAndLimit  SystemSampleTime=-1  VariantActivationTime=update diagram  Latency=0  AutoFrameSizeCalculation=off
      link override Signal_Limit/_maxval: Value=KOUTP_YawRateTimeOut_flg_maxval
      link override Signal_Limit/_minval: Value=KOUTP_YawRateTimeOut_flg_minval
      link override Signal_Override/_ovrdflg: Value=KOUTP_YawRateTimeOut_flg_ovrdflg
      link override Signal_Override/_ovrdval: Value=KOUTP_YawRateTimeOut_flg_ovrdval
  VAPM_YawRateVTimeOut_flg_Inproc : FVT_lib/outp/OverrideAndLimit  SystemSampleTime=-1  VariantActivationTime=update diagram  Latency=0  AutoFrameSizeCalculation=off
      link override Signal_Limit/_maxval: Value=KOUTP_YawRateVTimeOut_flg_maxval
      link override Signal_Limit/_minval: Value=KOUTP_YawRateVTimeOut_flg_minval
      link override Signal_Override/_ovrdflg: Value=KOUTP_YawRateVTimeOut_flg_ovrdflg
      link override Signal_Override/_ovrdval: Value=KOUTP_YawRateVTimeOut_flg_ovrdval
  VAPM_YawRateV_flg_Inproc : FVT_lib/outp/OverrideAndLimit  SystemSampleTime=-1  VariantActivationTime=update diagram  Latency=0  AutoFrameSizeCalculation=off
      link override Signal_Limit/_maxval: Value=KOUTP_YawRateV_flg_maxval
      link override Signal_Limit/_minval: Value=KOUTP_YawRateV_flg_minval
      link override Signal_Override/_ovrdflg: Value=KOUTP_YawRateV_flg_ovrdflg
      link override Signal_Override/_ovrdval: Value=KOUTP_YawRateV_flg_ovrdval
  VAPM_YawRate_degps_Inproc : FVT_lib/outp/OverrideAndLimit  SystemSampleTime=-1  VariantActivationTime=update diagram  Latency=0  AutoFrameSizeCalculation=off
      link override Signal_Limit/_maxval: Value=KOUTP_YawRate_degps_maxval
      link override Signal_Limit/_minval: Value=KOUTP_YawRate_degps_minval
      link override Signal_Override/_ovrdflg: Value=KOUTP_YawRate_degps_ovrdflg
      link override Signal_Override/_ovrdval: Value=KOUTP_YawRate_degps_ovrdval
  VBCM_BBuzzerCmd_flg_Inproc : FVT_lib/outp/OverrideAndLimit  SystemSampleTime=-1  VariantActivationTime=update diagram  Latency=0  AutoFrameSizeCalculation=off
      link override Signal_Limit/_maxval: Value=KOUTP_BBuzzerCmd_flg_maxval
      link override Signal_Limit/_minval: Value=KOUTP_BBuzzerCmd_flg_minval
      link override Signal_Override/_ovrdflg: Value=KOUTP_BBuzzerCmd_flg_ovrdflg
      link override Signal_Override/_ovrdval: Value=KOUTP_BBuzzerCmd_flg_ovrdval
  VBCM_BrakeLamp_flg_Inproc : FVT_lib/outp/OverrideAndLimit  SystemSampleTime=-1  VariantActivationTime=update diagram  Latency=0  AutoFrameSizeCalculation=off
      link override Signal_Limit/_maxval: Value=KOUTP_BrakeLamp_flg_maxval
      link override Signal_Limit/_minval: Value=KOUTP_BrakeLamp_flg_minval
      link override Signal_Override/_ovrdflg: Value=KOUTP_BrakeLamp_flg_ovrdflg
      link override Signal_Override/_ovrdval: Value=KOUTP_BrakeLamp_flg_ovrdval
  VBCM_DoorStaSta_enum_Inproc : FVT_lib/outp/OverrideAndLimit  SystemSampleTime=-1  VariantActivationTime=update diagram  Latency=0  AutoFrameSizeCalculation=off
      link override Signal_Limit/_maxval: Value=KOUTP_DoorStaSta_enum_maxval
      link override Signal_Limit/_minval: Value=KOUTP_DoorStaSta_enum_minval
      link override Signal_Override/_ovrdflg: Value=KOUTP_DoorStaSta_enum_ovrdflg
      link override Signal_Override/_ovrdval: Value=KOUTP_DoorStaSta_enum_ovrdval
  VBCM_FDDoorOpen_enum_Inproc : FVT_lib/outp/OverrideAndLimit  SystemSampleTime=-1  VariantActivationTime=update diagram  Latency=0  AutoFrameSizeCalculation=off
      link override Signal_Limit/_maxval: Value=KOUTP_FDDoorOpen_enum_maxval
      link override Signal_Limit/_minval: Value=KOUTP_FDDoorOpen_enum_minval
      link override Signal_Override/_ovrdflg: Value=KOUTP_FDDoorOpen_enum_ovrdflg
      link override Signal_Override/_ovrdval: Value=KOUTP_FDDoorOpen_enum_ovrdval
  VBCM_FDDoorstate_enum_Inproc : FVT_lib/outp/OverrideAndLimit  SystemSampleTime=-1  VariantActivationTime=update diagram  Latency=0  AutoFrameSizeCalculation=off
      link override Signal_Limit/_maxval: Value=KOUTP_FDDoorstate_enum_maxval
      link override Signal_Limit/_minval: Value=KOUTP_FDDoorstate_enum_minval
      link override Signal_Override/_ovrdflg: Value=KOUTP_FDDoorstate_enum_ovrdflg
      link override Signal_Override/_ovrdval: Value=KOUTP_FDDoorstate_enum_ovrdval
  VBCM_FRDisIntEmCmd_flg_Inproc : FVT_lib/outp/OverrideAndLimit  SystemSampleTime=-1  VariantActivationTime=update diagram  Latency=0  AutoFrameSizeCalculation=off
      link override Signal_Limit/_maxval: Value=KOUTP_FRDisIntEmCmd_flg_maxval
      link override Signal_Limit/_minval: Value=KOUTP_FRDisIntEmCmd_flg_minval
      link override Signal_Override/_ovrdflg: Value=KOUTP_FRDisIntEmCmd_flg_ovrdflg
      link override Signal_Override/_ovrdval: Value=KOUTP_FRDisIntEmCmd_flg_ovrdval
  VBCM_FRHaltBrakeSta_enum_Inproc : FVT_lib/outp/OverrideAndLimit  SystemSampleTime=-1  VariantActivationTime=update diagram  Latency=0  AutoFrameSizeCalculation=off
      link override Signal_Limit/_maxval: Value=KOUTP_FRHaltBrakeSta_enum_maxval
      link override Signal_Limit/_minval: Value=KOUTP_FRHaltBrakeSta_enum_minval
      link override Signal_Override/_ovrdflg: Value=KOUTP_FRHaltBrakeSta_enum_ovrdflg
      link override Signal_Override/_ovrdval: Value=KOUTP_FRHaltBrakeSta_enum_ovrdval
  VBCM_FROpenClosePBCmd_enum_Inproc : FVT_lib/outp/OverrideAndLimit  SystemSampleTime=-1  VariantActivationTime=update diagram  Latency=0  AutoFrameSizeCalculation=off
      link override Signal_Limit/_maxval: Value=KOUTP_FROpenClosePBCmd_enum_maxval
      link override Signal_Limit/_minval: Value=KOUTP_FROpenClosePBCmd_enum_minval
      link override Signal_Override/_ovrdflg: Value=KOUTP_FROpenClosePBCmd_enum_ovrdflg
      link override Signal_Override/_ovrdval: Value=KOUTP_FROpenClosePBCmd_enum_ovrdval
  VBCM_FrAtmoLampCmd_flg_Inproc : FVT_lib/outp/OverrideAndLimit  SystemSampleTime=-1  VariantActivationTime=update diagram  Latency=0  AutoFrameSizeCalculation=off
      link override Signal_Limit/_maxval: Value=KOUTP_FrAtmoLampCmd_flg_maxval
      link override Signal_Limit/_minval: Value=KOUTP_FrAtmoLampCmd_flg_minval
      link override Signal_Override/_ovrdflg: Value=KOUTP_FrAtmoLampCmd_flg_ovrdflg
      link override Signal_Override/_ovrdval: Value=KOUTP_FrAtmoLampCmd_flg_ovrdval
  VBCM_FrWiperH_flg_Inproc : FVT_lib/outp/OverrideAndLimit  SystemSampleTime=-1  VariantActivationTime=update diagram  Latency=0  AutoFrameSizeCalculation=off
      link override Signal_Limit/_maxval: Value=KOUTP_FrWiperH_flg_maxval
      link override Signal_Limit/_minval: Value=KOUTP_FrWiperH_flg_minval
      link override Signal_Override/_ovrdflg: Value=KOUTP_FrWiperH_flg_ovrdflg
      link override Signal_Override/_ovrdval: Value=KOUTP_FrWiperH_flg_ovrdval
  VBCM_FrWiperL_flg_Inproc : FVT_lib/outp/OverrideAndLimit  SystemSampleTime=-1  VariantActivationTime=update diagram  Latency=0  AutoFrameSizeCalculation=off
      link override Signal_Limit/_maxval: Value=KOUTP_FrWiperL_flg_maxval
      link override Signal_Limit/_minval: Value=KOUTP_FrWiperL_flg_minval
      link override Signal_Override/_ovrdflg: Value=KOUTP_FrWiperL_flg_ovrdflg
      link override Signal_Override/_ovrdval: Value=KOUTP_FrWiperL_flg_ovrdval
  VBCM_HBeam_flg_Inproc : FVT_lib/outp/OverrideAndLimit  SystemSampleTime=-1  VariantActivationTime=update diagram  Latency=0  AutoFrameSizeCalculation=off
      link override Signal_Limit/_maxval: Value=KOUTP_HBeam_flg_maxval
      link override Signal_Limit/_minval: Value=KOUTP_HBeam_flg_minval
      link override Signal_Override/_ovrdflg: Value=KOUTP_HBeam_flg_ovrdflg
      link override Signal_Override/_ovrdval: Value=KOUTP_HBeam_flg_ovrdval
  VBCM_HazardSW_flg_Inproc : FVT_lib/outp/OverrideAndLimit  SystemSampleTime=-1  VariantActivationTime=update diagram  Latency=0  AutoFrameSizeCalculation=off
      link override Signal_Limit/_maxval: Value=KOUTP_HazardSW_flg_maxval
      link override Signal_Limit/_minval: Value=KOUTP_HazardSW_flg_minval
      link override Signal_Override/_ovrdflg: Value=KOUTP_HazardSW_flg_ovrdflg
      link override Signal_Override/_ovrdval: Value=KOUTP_HazardSW_flg_ovrdval
  VBCM_HornCtrl_flg_Inproc : FVT_lib/outp/OverrideAndLimit  SystemSampleTime=-1  VariantActivationTime=update diagram  Latency=0  AutoFrameSizeCalculation=off
      link override Signal_Limit/_maxval: Value=KOUTP_HornCtrl_flg_maxval
      link override Signal_Limit/_minval: Value=KOUTP_HornCtrl_flg_minval
      link override Signal_Override/_ovrdflg: Value=KOUTP_HornCtrl_flg_ovrdflg
      link override Signal_Override/_ovrdval: Value=KOUTP_HornCtrl_flg_ovrdval
  VBCM_LBeam_flg_Inproc : FVT_lib/outp/OverrideAndLimit  SystemSampleTime=-1  VariantActivationTime=update diagram  Latency=0  AutoFrameSizeCalculation=off
      link override Signal_Limit/_maxval: Value=KOUTP_LBeam_flg_maxval
      link override Signal_Limit/_minval: Value=KOUTP_LBeam_flg_minval
      link override Signal_Override/_ovrdflg: Value=KOUTP_LBeam_flg_ovrdflg
      link override Signal_Override/_ovrdval: Value=KOUTP_LBeam_flg_ovrdval
  VBCM_LDRL_flg_Inproc : FVT_lib/outp/OverrideAndLimit  SystemSampleTime=-1  VariantActivationTime=update diagram  Latency=0  AutoFrameSizeCalculation=off
      link override Signal_Limit/_maxval: Value=KOUTP_LDRL_flg_maxval
      link override Signal_Limit/_minval: Value=KOUTP_LDRL_flg_minval
      link override Signal_Override/_ovrdflg: Value=KOUTP_LDRL_flg_ovrdflg
      link override Signal_Override/_ovrdval: Value=KOUTP_LDRL_flg_ovrdval
  VBCM_LSMLPCmd_flg_Inproc : FVT_lib/outp/OverrideAndLimit  SystemSampleTime=-1  VariantActivationTime=update diagram  Latency=0  AutoFrameSizeCalculation=off
      link override Signal_Limit/_maxval: Value=KOUTP_LSMLPCmd_flg_maxval
      link override Signal_Limit/_minval: Value=KOUTP_LSMLPCmd_flg_minval
      link override Signal_Override/_ovrdflg: Value=KOUTP_LSMLPCmd_flg_ovrdflg
      link override Signal_Override/_ovrdval: Value=KOUTP_LSMLPCmd_flg_ovrdval
  VBCM_LTgateRelCmd_flg_Inproc : FVT_lib/outp/OverrideAndLimit  SystemSampleTime=-1  VariantActivationTime=update diagram  Latency=0  AutoFrameSizeCalculation=off
      link override Signal_Limit/_maxval: Value=KOUTP_LTgateRelCmd_flg_maxval
      link override Signal_Limit/_minval: Value=KOUTP_LTgateRelCmd_flg_minval
      link override Signal_Override/_ovrdflg: Value=KOUTP_LTgateRelCmd_flg_ovrdflg
      link override Signal_Override/_ovrdval: Value=KOUTP_LTgateRelCmd_flg_ovrdval
  VBCM_LTurnLP_flg_Inproc : FVT_lib/outp/OverrideAndLimit  SystemSampleTime=-1  VariantActivationTime=update diagram  Latency=0  AutoFrameSizeCalculation=off
      link override Signal_Limit/_maxval: Value=KOUTP_LTurnLP_flg_maxval
      link override Signal_Limit/_minval: Value=KOUTP_LTurnLP_flg_minval
      link override Signal_Override/_ovrdflg: Value=KOUTP_LTurnLP_flg_ovrdflg
      link override Signal_Override/_ovrdval: Value=KOUTP_LTurnLP_flg_ovrdval
  VBCM_PosLamp_flg_Inproc : FVT_lib/outp/OverrideAndLimit  SystemSampleTime=-1  VariantActivationTime=update diagram  Latency=0  AutoFrameSizeCalculation=off
      link override Signal_Limit/_maxval: Value=KOUTP_PosLamp_flg_maxval
      link override Signal_Limit/_minval: Value=KOUTP_PosLamp_flg_minval
      link override Signal_Override/_ovrdflg: Value=KOUTP_PosLamp_flg_ovrdflg
      link override Signal_Override/_ovrdval: Value=KOUTP_PosLamp_flg_ovrdval
  VBCM_RDRL_flg_Inproc : FVT_lib/outp/OverrideAndLimit  SystemSampleTime=-1  VariantActivationTime=update diagram  Latency=0  AutoFrameSizeCalculation=off
      link override Signal_Limit/_maxval: Value=KOUTP_RDRL_flg_maxval
      link override Signal_Limit/_minval: Value=KOUTP_RDRL_flg_minval
      link override Signal_Override/_ovrdflg: Value=KOUTP_RDRL_flg_ovrdflg
      link override Signal_Override/_ovrdval: Value=KOUTP_RDRL_flg_ovrdval
  VBCM_RSMLPCmd_flg_Inproc : FVT_lib/outp/OverrideAndLimit  SystemSampleTime=-1  VariantActivationTime=update diagram  Latency=0  AutoFrameSizeCalculation=off
      link override Signal_Limit/_maxval: Value=KOUTP_RSMLPCmd_flg_maxval
      link override Signal_Limit/_minval: Value=KOUTP_RSMLPCmd_flg_minval
      link override Signal_Override/_ovrdflg: Value=KOUTP_RSMLPCmd_flg_ovrdflg
      link override Signal_Override/_ovrdval: Value=KOUTP_RSMLPCmd_flg_ovrdval
  VBCM_RTgateRelCmd_flg_Inproc : FVT_lib/outp/OverrideAndLimit  SystemSampleTime=-1  VariantActivationTime=update diagram  Latency=0  AutoFrameSizeCalculation=off
      link override Signal_Limit/_maxval: Value=KOUTP_RTgateRelCmd_flg_maxval
      link override Signal_Limit/_minval: Value=KOUTP_RTgateRelCmd_flg_minval
      link override Signal_Override/_ovrdflg: Value=KOUTP_RTgateRelCmd_flg_ovrdflg
      link override Signal_Override/_ovrdval: Value=KOUTP_RTgateRelCmd_flg_ovrdval
  VBCM_RTurnLP_flg_Inproc : FVT_lib/outp/OverrideAndLimit  SystemSampleTime=-1  VariantActivationTime=update diagram  Latency=0  AutoFrameSizeCalculation=off
      link override Signal_Limit/_maxval: Value=KOUTP_RTurnLP_flg_maxval
      link override Signal_Limit/_minval: Value=KOUTP_RTurnLP_flg_minval
      link override Signal_Override/_ovrdflg: Value=KOUTP_RTurnLP_flg_ovrdflg
      link override Signal_Override/_ovrdval: Value=KOUTP_RTurnLP_flg_ovrdval
  VBCM_ReverseLamp_flg_Inproc : FVT_lib/outp/OverrideAndLimit  SystemSampleTime=-1  VariantActivationTime=update diagram  Latency=0  AutoFrameSizeCalculation=off
      link override Signal_Limit/_maxval: Value=KOUTP_ReverseLamp_flg_maxval
      link override Signal_Limit/_minval: Value=KOUTP_ReverseLamp_flg_minval
      link override Signal_Override/_ovrdflg: Value=KOUTP_ReverseLamp_flg_ovrdflg
      link override Signal_Override/_ovrdval: Value=KOUTP_ReverseLamp_flg_ovrdval
  VBCM_RrAtmoLampCmd_flg_Inproc : FVT_lib/outp/OverrideAndLimit  SystemSampleTime=-1  VariantActivationTime=update diagram  Latency=0  AutoFrameSizeCalculation=off
      link override Signal_Limit/_maxval: Value=KOUTP_RrAtmoLampCmd_flg_maxval
      link override Signal_Limit/_minval: Value=KOUTP_RrAtmoLampCmd_flg_minval
      link override Signal_Override/_ovrdflg: Value=KOUTP_RrAtmoLampCmd_flg_ovrdflg
      link override Signal_Override/_ovrdval: Value=KOUTP_RrAtmoLampCmd_flg_ovrdval
  VBCM_RrFogLamp_flg_Inproc : FVT_lib/outp/OverrideAndLimit  SystemSampleTime=-1  VariantActivationTime=update diagram  Latency=0  AutoFrameSizeCalculation=off
      link override Signal_Limit/_maxval: Value=KOUTP_RrFogLamp_flg_maxval
      link override Signal_Limit/_minval: Value=KOUTP_RrFogLamp_flg_minval
      link override Signal_Override/_ovrdflg: Value=KOUTP_RrFogLamp_flg_ovrdflg
      link override Signal_Override/_ovrdval: Value=KOUTP_RrFogLamp_flg_ovrdval
  VBCM_RrRmLampBrightCmd_enum_Inproc : FVT_lib/outp/OverrideAndLimit  SystemSampleTime=-1  VariantActivationTime=update diagram  Latency=0  AutoFrameSizeCalculation=off
      link override Signal_Limit/_maxval: Value=KOUTP_RrRmLampBrightCmd_enum_maxval
      link override Signal_Limit/_minval: Value=KOUTP_RrRmLampBrightCmd_enum_minval
      link override Signal_Override/_ovrdflg: Value=KOUTP_RrRmLampBrightCmd_enum_ovrdflg
      link override Signal_Override/_ovrdval: Value=KOUTP_RrRmLampBrightCmd_enum_ovrdval
  VBCM_TgateHDSWLSta_flg_Inproc : FVT_lib/outp/OverrideAndLimit  SystemSampleTime=-1  VariantActivationTime=update diagram  Latency=0  AutoFrameSizeCalculation=off
      link override Signal_Limit/_maxval: Value=KOUTP_TgateHDSWLSta_flg_maxval
      link override Signal_Limit/_minval: Value=KOUTP_TgateHDSWLSta_flg_minval
      link override Signal_Override/_ovrdflg: Value=KOUTP_TgateHDSWLSta_flg_ovrdflg
      link override Signal_Override/_ovrdval: Value=KOUTP_TgateHDSWLSta_flg_ovrdval
  VBCM_TgateHDSWRSta_flg_Inproc : FVT_lib/outp/OverrideAndLimit  SystemSampleTime=-1  VariantActivationTime=update diagram  Latency=0  AutoFrameSizeCalculation=off
      link override Signal_Limit/_maxval: Value=KOUTP_TgateHDSWRSta_flg_maxval
      link override Signal_Limit/_minval: Value=KOUTP_TgateHDSWRSta_flg_minval
      link override Signal_Override/_ovrdflg: Value=KOUTP_TgateHDSWRSta_flg_ovrdflg
      link override Signal_Override/_ovrdval: Value=KOUTP_TgateHDSWRSta_flg_ovrdval
  VBCM_TgateSWLSta_flg_Inproc : FVT_lib/outp/OverrideAndLimit  SystemSampleTime=-1  VariantActivationTime=update diagram  Latency=0  AutoFrameSizeCalculation=off
      link override Signal_Limit/_maxval: Value=KOUTP_TgateSWLSta_flg_maxval
      link override Signal_Limit/_minval: Value=KOUTP_TgateSWLSta_flg_minval
      link override Signal_Override/_ovrdflg: Value=KOUTP_TgateSWLSta_flg_ovrdflg
      link override Signal_Override/_ovrdval: Value=KOUTP_TgateSWLSta_flg_ovrdval
  VBCM_TgateSWRSta_flg_Inproc : FVT_lib/outp/OverrideAndLimit  SystemSampleTime=-1  VariantActivationTime=update diagram  Latency=0  AutoFrameSizeCalculation=off
      link override Signal_Limit/_maxval: Value=KOUTP_TgateSWRSta_flg_maxval
      link override Signal_Limit/_minval: Value=KOUTP_TgateSWRSta_flg_minval
      link override Signal_Override/_ovrdflg: Value=KOUTP_TgateSWRSta_flg_ovrdflg
      link override Signal_Override/_ovrdval: Value=KOUTP_TgateSWRSta_flg_ovrdval
  VBCM_TurnLpLActiveCmd_flg_Inproc : FVT_lib/outp/OverrideAndLimit  SystemSampleTime=-1  VariantActivationTime=update diagram  Latency=0  AutoFrameSizeCalculation=off
      link override Signal_Limit/_maxval: Value=KOUTP_TurnLpLActiveCmd_flg_maxval
      link override Signal_Limit/_minval: Value=KOUTP_TurnLpLActiveCmd_flg_minval
      link override Signal_Override/_ovrdflg: Value=KOUTP_TurnLpLActiveCmd_flg_ovrdflg
      link override Signal_Override/_ovrdval: Value=KOUTP_TurnLpLActiveCmd_flg_ovrdval
  VBCM_TurnLpRActiveCmd_flg_Inproc : FVT_lib/outp/OverrideAndLimit  SystemSampleTime=-1  VariantActivationTime=update diagram  Latency=0  AutoFrameSizeCalculation=off
      link override Signal_Limit/_maxval: Value=KOUTP_TurnLpRActiveCmd_flg_maxval
      link override Signal_Limit/_minval: Value=KOUTP_TurnLpRActiveCmd_flg_minval
      link override Signal_Override/_ovrdflg: Value=KOUTP_TurnLpRActiveCmd_flg_ovrdflg
      link override Signal_Override/_ovrdval: Value=KOUTP_TurnLpRActiveCmd_flg_ovrdval
  VBCM_WasherCtrl_enum_Inproc : FVT_lib/outp/OverrideAndLimit  SystemSampleTime=-1  VariantActivationTime=update diagram  Latency=0  AutoFrameSizeCalculation=off
      link override Signal_Limit/_maxval: Value=KOUTP_WasherCtrl_enum_maxval
      link override Signal_Limit/_minval: Value=KOUTP_WasherCtrl_enum_minval
      link override Signal_Override/_ovrdflg: Value=KOUTP_WasherCtrl_enum_ovrdflg
      link override Signal_Override/_ovrdval: Value=KOUTP_WasherCtrl_enum_ovrdval
  VBCM_WelcomeDemoSta_flg_Inproc : FVT_lib/outp/OverrideAndLimit  SystemSampleTime=-1  VariantActivationTime=update diagram  Latency=0  AutoFrameSizeCalculation=off
      link override Signal_Limit/_maxval: Value=KOUTP_WelcomeDemoSta_flg_maxval
      link override Signal_Limit/_minval: Value=KOUTP_WelcomeDemoSta_flg_minval
      link override Signal_Override/_ovrdflg: Value=KOUTP_WelcomeDemoSta_flg_ovrdflg
      link override Signal_Override/_ovrdval: Value=KOUTP_WelcomeDemoSta_flg_ovrdval
  VDHP_ActAPSPosn_pct_Inproc : FVT_lib/outp/OverrideAndLimit  SystemSampleTime=-1  VariantActivationTime=update diagram  Latency=0  AutoFrameSizeCalculation=off
      link override Signal_Limit/_maxval: Value=KOUTP_ActAPSPosn_pct_maxval
      link override Signal_Limit/_minval: Value=KOUTP_ActAPSPosn_pct_minval
      link override Signal_Override/_ovrdflg: Value=KOUTP_ActAPSPosn_pct_ovrdflg
      link override Signal_Override/_ovrdval: Value=KOUTP_ActAPSPosn_pct_ovrdval
  VDHP_EAPS1MIN_pct_Inproc : FVT_lib/outp/OverrideAndLimit  SystemSampleTime=-1  VariantActivationTime=update diagram  Latency=0  AutoFrameSizeCalculation=off
      link override Signal_Limit/_maxval: Value=KOUTP_EAPS1MIN_pct_maxval
      link override Signal_Limit/_minval: Value=KOUTP_EAPS1MIN_pct_minval
      link override Signal_Override/_ovrdflg: Value=KOUTP_EAPS1MIN_pct_ovrdflg
      link override Signal_Override/_ovrdval: Value=KOUTP_EAPS1MIN_pct_ovrdval
  VDHP_EAPS2MIN_pct_Inproc : FVT_lib/outp/OverrideAndLimit  SystemSampleTime=-1  VariantActivationTime=update diagram  Latency=0  AutoFrameSizeCalculation=off
      link override Signal_Limit/_maxval: Value=KOUTP_EAPS2MIN_pct_maxval
      link override Signal_Limit/_minval: Value=KOUTP_EAPS2MIN_pct_minval
      link override Signal_Override/_ovrdflg: Value=KOUTP_EAPS2MIN_pct_ovrdflg
      link override Signal_Override/_ovrdval: Value=KOUTP_EAPS2MIN_pct_ovrdval
  VDKC_DKCAuthSta_enum_Inproc : FVT_lib/outp/OverrideAndLimit  SystemSampleTime=-1  VariantActivationTime=update diagram  Latency=0  AutoFrameSizeCalculation=off
      link override Signal_Limit/_maxval: Value=KOUTP_DKCAuthSta_enum_maxval
      link override Signal_Limit/_minval: Value=KOUTP_DKCAuthSta_enum_minval
      link override Signal_Override/_ovrdflg: Value=KOUTP_DKCAuthSta_enum_ovrdflg
      link override Signal_Override/_ovrdval: Value=KOUTP_DKCAuthSta_enum_ovrdval
  VDKC_DKCTimeSN_cnt_Inproc : FVT_lib/outp/OverrideAndLimit  SystemSampleTime=-1  VariantActivationTime=update diagram  Latency=0  AutoFrameSizeCalculation=off
      link override Signal_Limit/_maxval: Value=KOUTP_DKCTimeSN_cnt_maxval
      link override Signal_Limit/_minval: Value=KOUTP_DKCTimeSN_cnt_minval
      link override Signal_Override/_ovrdflg: Value=KOUTP_DKCTimeSN_cnt_ovrdflg
      link override Signal_Override/_ovrdval: Value=KOUTP_DKCTimeSN_cnt_ovrdval
  VDSC_DISCButtSta_flg_Inproc : FVT_lib/outp/OverrideAndLimit  SystemSampleTime=-1  VariantActivationTime=update diagram  Latency=0  AutoFrameSizeCalculation=off
      link override Signal_Limit/_maxval: Value=KOUTP_DISCButtSta_flg_maxval
      link override Signal_Limit/_minval: Value=KOUTP_DISCButtSta_flg_minval
      link override Signal_Override/_ovrdflg: Value=KOUTP_DISCButtSta_flg_ovrdflg
      link override Signal_Override/_ovrdval: Value=KOUTP_DISCButtSta_flg_ovrdval
  VDSC_DISCSta_enum_Inproc : FVT_lib/outp/OverrideAndLimit  SystemSampleTime=-1  VariantActivationTime=update diagram  Latency=0  AutoFrameSizeCalculation=off
      link override Signal_Limit/_maxval: Value=KOUTP_DISCSta_enum_maxval
      link override Signal_Limit/_minval: Value=KOUTP_DISCSta_enum_minval
      link override Signal_Override/_ovrdflg: Value=KOUTP_DISCSta_enum_ovrdflg
      link override Signal_Override/_ovrdval: Value=KOUTP_DISCSta_enum_ovrdval
  VDSC_DISCTargetSpd_kph_Inproc : FVT_lib/outp/OverrideAndLimit  SystemSampleTime=-1  VariantActivationTime=update diagram  Latency=0  AutoFrameSizeCalculation=off
      link override Signal_Limit/_maxval: Value=KOUTP_DISCTargetSpd_kph_maxval
      link override Signal_Limit/_minval: Value=KOUTP_DISCTargetSpd_kph_minval
      link override Signal_Override/_ovrdflg: Value=KOUTP_DISCTargetSpd_kph_ovrdflg
      link override Signal_Override/_ovrdval: Value=KOUTP_DISCTargetSpd_kph_ovrdval
  VDSC_DISCTurn_flg_Inproc : FVT_lib/outp/OverrideAndLimit  SystemSampleTime=-1  VariantActivationTime=update diagram  Latency=0  AutoFrameSizeCalculation=off
      link override Signal_Limit/_maxval: Value=KOUTP_DISCTurn_flg_maxval
      link override Signal_Limit/_minval: Value=KOUTP_DISCTurn_flg_minval
      link override Signal_Override/_ovrdflg: Value=KOUTP_DISCTurn_flg_ovrdflg
      link override Signal_Override/_ovrdval: Value=KOUTP_DISCTurn_flg_ovrdval
  VNMM_ActiveWU_flg_Inproc : FVT_lib/outp/OverrideAndLimit  SystemSampleTime=-1  VariantActivationTime=update diagram  Latency=0  AutoFrameSizeCalculation=off
      link override Signal_Limit/_maxval: Value=KOUTP_ActiveWU_flg_maxval
      link override Signal_Limit/_minval: Value=KOUTP_ActiveWU_flg_minval
      link override Signal_Override/_ovrdflg: Value=KOUTP_ActiveWU_flg_ovrdflg
      link override Signal_Override/_ovrdval: Value=KOUTP_ActiveWU_flg_ovrdval
  VNMM_AllCANTxReq_flg_Inproc : FVT_lib/outp/OverrideAndLimit  SystemSampleTime=-1  VariantActivationTime=update diagram  Latency=0  AutoFrameSizeCalculation=off
      link override Signal_Limit/_maxval: Value=KOUTP_AllCANTxReq_flg_maxval
      link override Signal_Limit/_minval: Value=KOUTP_AllCANTxReq_flg_minval
      link override Signal_Override/_ovrdflg: Value=KOUTP_AllCANTxReq_flg_ovrdflg
      link override Signal_Override/_ovrdval: Value=KOUTP_AllCANTxReq_flg_ovrdval
  VNMM_Awake_enum_Inproc : FVT_lib/outp/OverrideAndLimit  SystemSampleTime=-1  VariantActivationTime=update diagram  Latency=0  AutoFrameSizeCalculation=off
      link override Signal_Limit/_maxval: Value=KOUTP_Awake_enum_maxval
      link override Signal_Limit/_minval: Value=KOUTP_Awake_enum_minval
      link override Signal_Override/_ovrdflg: Value=KOUTP_Awake_enum_ovrdflg
      link override Signal_Override/_ovrdval: Value=KOUTP_Awake_enum_ovrdval
  VNMM_CSB_flg_Inproc : FVT_lib/outp/OverrideAndLimit  SystemSampleTime=-1  VariantActivationTime=update diagram  Latency=0  AutoFrameSizeCalculation=off
      link override Signal_Limit/_maxval: Value=KOUTP_CSB_flg_maxval
      link override Signal_Limit/_minval: Value=KOUTP_CSB_flg_minval
      link override Signal_Override/_ovrdflg: Value=KOUTP_CSB_flg_ovrdflg
      link override Signal_Override/_ovrdval: Value=KOUTP_CSB_flg_ovrdval
  VNMM_ErrorState_enum_Inproc : FVT_lib/outp/OverrideAndLimit  SystemSampleTime=-1  VariantActivationTime=update diagram  Latency=0  AutoFrameSizeCalculation=off
      link override Signal_Limit/_maxval: Value=KOUTP_ErrorState_enum_maxval
      link override Signal_Limit/_minval: Value=KOUTP_ErrorState_enum_minval
      link override Signal_Override/_ovrdflg: Value=KOUTP_ErrorState_enum_ovrdflg
      link override Signal_Override/_ovrdval: Value=KOUTP_ErrorState_enum_ovrdval
  VNMM_NMmTxReq_flg_Inproc : FVT_lib/outp/OverrideAndLimit  SystemSampleTime=-1  VariantActivationTime=update diagram  Latency=0  AutoFrameSizeCalculation=off
      link override Signal_Limit/_maxval: Value=KOUTP_NMmTxReq_flg_maxval
      link override Signal_Limit/_minval: Value=KOUTP_NMmTxReq_flg_minval
      link override Signal_Override/_ovrdflg: Value=KOUTP_NMmTxReq_flg_ovrdflg
      link override Signal_Override/_ovrdval: Value=KOUTP_NMmTxReq_flg_ovrdval
  VNMM_NetworkReq_flg_Inproc : FVT_lib/outp/OverrideAndLimit  SystemSampleTime=-1  VariantActivationTime=update diagram  Latency=0  AutoFrameSizeCalculation=off
      link override Signal_Limit/_maxval: Value=KOUTP_NetworkReq_flg_maxval
      link override Signal_Limit/_minval: Value=KOUTP_NetworkReq_flg_minval
      link override Signal_Override/_ovrdflg: Value=KOUTP_NetworkReq_flg_ovrdflg
      link override Signal_Override/_ovrdval: Value=KOUTP_NetworkReq_flg_ovrdval
  VNMM_NodeID_enum_Inproc : FVT_lib/outp/OverrideAndLimit  SystemSampleTime=-1  VariantActivationTime=update diagram  Latency=0  AutoFrameSizeCalculation=off
      link override Signal_Limit/_maxval: Value=KOUTP_NodeID_enum_maxval
      link override Signal_Limit/_minval: Value=KOUTP_NodeID_enum_minval
      link override Signal_Override/_ovrdflg: Value=KOUTP_NodeID_enum_ovrdflg
      link override Signal_Override/_ovrdval: Value=KOUTP_NodeID_enum_ovrdval
  VNMM_PNI_flg_Inproc : FVT_lib/outp/OverrideAndLimit  SystemSampleTime=-1  VariantActivationTime=update diagram  Latency=0  AutoFrameSizeCalculation=off
      link override Signal_Limit/_maxval: Value=KOUTP_PNI_flg_maxval
      link override Signal_Limit/_minval: Value=KOUTP_PNI_flg_minval
      link override Signal_Override/_ovrdflg: Value=KOUTP_PNI_flg_ovrdflg
      link override Signal_Override/_ovrdval: Value=KOUTP_PNI_flg_ovrdval
  VNMM_RptMsgReq_flg_Inproc : FVT_lib/outp/OverrideAndLimit  SystemSampleTime=-1  VariantActivationTime=update diagram  Latency=0  AutoFrameSizeCalculation=off
      link override Signal_Limit/_maxval: Value=KOUTP_RptMsgReq_flg_maxval
      link override Signal_Limit/_minval: Value=KOUTP_RptMsgReq_flg_minval
      link override Signal_Override/_ovrdflg: Value=KOUTP_RptMsgReq_flg_ovrdflg
      link override Signal_Override/_ovrdval: Value=KOUTP_RptMsgReq_flg_ovrdval
  VNMM_SysNMmSta_enum_Inproc : FVT_lib/outp/OverrideAndLimit  SystemSampleTime=-1  VariantActivationTime=update diagram  Latency=0  AutoFrameSizeCalculation=off
      link override Signal_Limit/_maxval: Value=KOUTP_SysNMmSta_enum_maxval
      link override Signal_Limit/_minval: Value=KOUTP_SysNMmSta_enum_minval
      link override Signal_Override/_ovrdflg: Value=KOUTP_SysNMmSta_enum_ovrdflg
      link override Signal_Override/_ovrdval: Value=KOUTP_SysNMmSta_enum_ovrdval
  VNMM_WakeUp_enum_Inproc : FVT_lib/outp/OverrideAndLimit  SystemSampleTime=-1  VariantActivationTime=update diagram  Latency=0  AutoFrameSizeCalculation=off
      link override Signal_Limit/_maxval: Value=KOUTP_WakeUp_enum_maxval
      link override Signal_Limit/_minval: Value=KOUTP_WakeUp_enum_minval
      link override Signal_Override/_ovrdflg: Value=KOUTP_WakeUp_enum_ovrdflg
      link override Signal_Override/_ovrdval: Value=KOUTP_WakeUp_enum_ovrdval
